simulink model "bus_roadtest_v3"  (R2018a)
settings: Solver=ode3  StartTime=0.0  StopTime=inf  FixedStep=0.01  RelTol=1e-3  EnableMultiTasking=on
PostLoadFcn:
  | , if any(exist('dsrtsu_mdlpostloadfcn', 'file') == [2, 3, 6]), try dsrtsu_mdlpostloadfcn('Execute', bdroot); catch fprintf('Error in PostLoadFcn (dsrtsu_mdlpostloadfcn) for model "%s":\n %s\n', bdroot, lasterr); end, end,
InitFcn:
  | bus_roadtest_v3_initial
values from neighbouring files (symbols this model uses):
  ay_max = 2    [Ini.m]
  delta_t = 0.01    [Ini.m]
  end_left_pass = 1    [Ini.m]
  end_right_pass = 0    [Ini.m]
  finish_node_id = length(Map_data(:,1))    [Ini.m]
  forward_length = 15    [Ini.m]
  gamma = sqrt(N_xaug+lambda)    [bus_roadtest_v3_initial.m]
  k_safe = 1    [Ini.m]
  nodes = nodes(1:index_node,:)    [Ini.m]
  rmin = 10    [Ini.m]
  segments = zeros(length(xy_ends_Pos(:,1)),3)    [Ini.m]
  start_node_id = 1    [Ini.m]
  Ts = 0.01    [bus_roadtest_v3_initial.m]
  Veh_CG = [0.5, 0.2]    [Ini.m]
  Veh_size = [1.99986,6.09558]    [Ini.m]
  vmax = 6    [Ini.m]
  weight = [weight_0,weight_0_cov,weight_i]    [bus_roadtest_v3_initial.m]
undefined symbols (not defined in the file or in its folder): Brake_table, DiscIntNeverNeededParam, Map_data, R, REF_GPS_RFS, Steer_gain_table, T
libraries: rtican x71, simulink x26, rti1401lib_adc_type4 x8, rti1401lib_dio_type4 x1
(part 7 of 18)

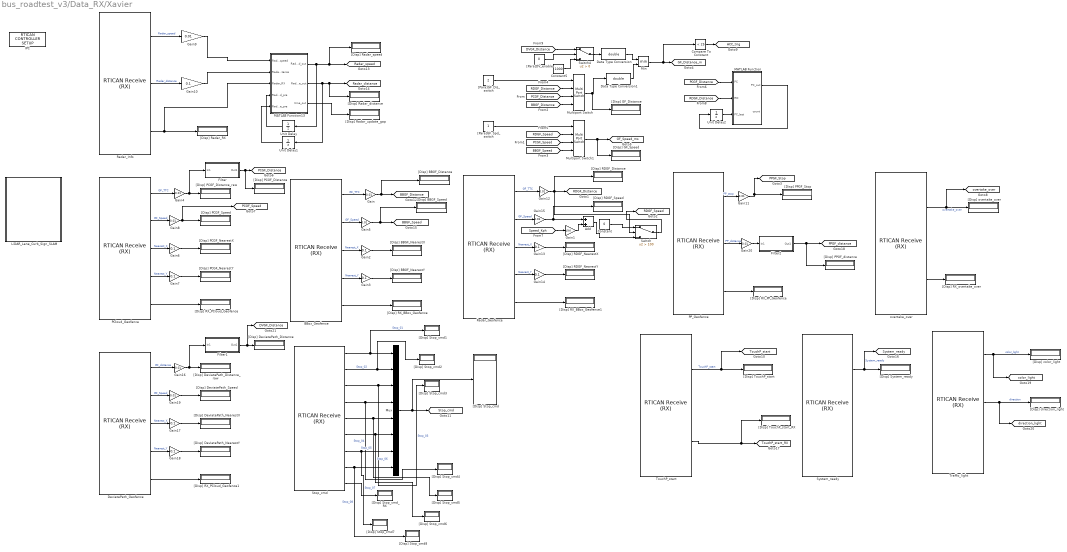
== system bus_roadtest_v3/Data_RX/Xavier ==
  Add : Sum
  BBox_Geofence : rtican/RTICAN Receive (RX)   Reserved1=[]  Reserved2=[]  Reserved3=[]  Reserved4=[]  SfcnMessage=[]  Msg_Struct=[]  BoardTypeNo=[]  BoardNo=[]  ChannelNo=[]  Parameters=[]  DialogFcn=[]  UnitName=[]  Revision=[]  UnitValues=[]  DSProperties=struct('RTI',struct('Version',uint32(5),'BlockType',struct('isSLSource',uint8(1),'isSLSink',uint8(1),'isHWSource',uint8(0),'isHWSink',uint8(0),'isSetup',uint8(0),'isInline',uint8(1),'isNonInline',uint8(0),'isInterrupt',uint8(0),'isChannelwise',uint8(0)),'IOBoardType','RTICAN','UnitType','MESSAGE','Identifier','RX','DialogType','MSVC','BlockSet','RTICAN','SlaveProcessor','CAN'))  RTIBlockInterface=struct('OutputPortsWidth',int32([1 1 1 1 1]),'OutputPortsActive',[1 1 1 1 1],'OutputPortsName',{{'GF_TTC','GF_Speed','Nearest_X','Nearest_Y',['RX status']}},'OutputPortsDataType',{{'SS_DOUBLE','SS_DOUBLE','SS_DOUBLE','SS_DOUBLE','SS_DOUBLE'}},'OutputPortsLabel',{{'GF_TTC','GF_Speed','Nearest_X','Nearest_Y',''}},'OutputPortsLabelMode','ON','InputPortsWidth',int32(0),'InputPortsActive',0,'DialogFcn','rtican_message_interface_gui','BlockDisplay',{{'','center'}},'IconTransparency','on','ParameterTunableNames',{{}},'InitLevel',3,'BlockName',struct('Token',{{'Geo_Fence_msg1'}}),'SampleTime',{{-1}},'TriggerPort',{{'none'}},'EnablePort',{{'none'}})  RTIBlockParameters=struct('BoardTypeNo',{{1,'OFF',[]}},'BoardNo',{{1,'ON',[1 16]}},'ChannelNo',{{1,'ON',[1 2]}},'Parameters',{{struct('DataFileSupport',struct('DataFileSelectedMaster',0,'DataFileSelectedLocal',0,'DataFileName',['<no datafile support>|'],'DataFileDate','','SelectedFile',['<no file selected>']),'Options',struct('StatusSelected',1,'TimeSelected',0,'DeltaTimeSelected',0,'BytePortSelected',0,'MessageLengthSelected',0,'TriggerPort',struct('Selected',0,'TriggerType',0),'UserCoding',struct('Selected',0,'InterfaceFile','UserDecodingFile','FcnName','UserDecodeFcn','InportSelected',0,'InportWidth',1,'OutportSelected',0,'OutportWidth',1),'EnablePortSelected',0,'SignalOnPortnameSelected',1,'UseRXService',0),'Message',struct('MsgOnBlocknameSelected',1,'MsgName','BBox_Geofence','MsgIdFormat',0,'MsgId',1425,'MsgLength',8,'NumSignals',4,'SampleTime',-1,'Signal',struct('SgnName',{'GF_TTC','GF_Speed','Nearest_X','Nearest_Y'},'SgnStartBit',{0,16,32,48},'SgnLength',{16,16,16,16},'SgnType',{0,0,0,0},'ModeValue',{-1,-1,-1,-1},'DataType',{1,1,1,1},'ByteLayout',{0,0,0,0},'Factor',{1,1,1,1},'Offset',{0,0,0,0},'SgnComment',{{''},{''},{''},{''}},'SgnUnit',{'','','',''},'Min',{0,0,0,0},'Max',{0,0,0,0},'SLDataType',{'SS_DOUBLE','SS_DOUBLE','SS_DOUBLE','SS_DOUBLE'}),'MsgIdNumFormat',1,'MsgComment',{{''}}),'Version',1.2,'general',struct('isFromLib',0)),'OFF',[]}},'GroupId',{{struct('Group',{{'RTICAN'}},'No',2,'Behavior',{{'NAMECHANGE'}},'BlockType',{{'SINK'}},'NameChangeFlag',0),'OFF',[]}},'SFcnRTICANMessage',{{struct('MsgType','RX','SFcnPortType','Scalar','MsgName','BBox_Geofence','MsgIdFormat','STD','MsgId',1425,'MsgLength',8,'NumSignals',4,'SampleTime',-1,'Signal',struct('SgnName',{'GF_TTC','GF_Speed','Nearest_X','Nearest_Y'},'SgnStartBit',{0,16,32,48},'SgnLength',{16,16,16,16},'SgnType',{'standard','standard','standard','standard'},'ModeValue',{-1,-1,-1,-1},'DataType',{['signed int'],['signed int'],['signed int'],['signed int']},'ByteLayout',{['little endian'],['little endian'],['little endian'],['little endian']},'Factor',{1,1,1,1},'Offset',{0,0,0,0},'SLDataType',{'SS_DOUBLE','SS_DOUBLE','SS_DOUBLE','SS_DOUBLE'}),'StatusSelected','yes','TimeSelected','no','DeltaTimeSelected','no','BytePortSelected','no','MessageLengthSelected','no','TriggerPort',struct('Selected','no','TriggerType',0),'UserCoding',struct('Selected','no','InterfaceFile','UserDecodingFile','FcnName','UserDecodeFcn','InportSelected','no','InportWidth',1,'OutportSelected','no','OutportWidth',1),'EnablePortSelected','no','UseRXService','no','BoardType','DS1','BoardNo',1,'ControllerNo',1),'OFF',[]}},'TLCFileName',{{'rtican_rx_message','OFF',[]}})  RTISFcnParameters=struct('SFcnRTICANMessage','struct','TLCFileName','char')  RTIBlockParaDefault=struct('BoardTypeNo',4302,'BoardNo',1,'ChannelNo',1,'Parameters',struct('DataFileSupport',struct('DataFileSelectedMaster',0,'DataFileSelectedLocal',0,'DataFileName','','DataFileDate','','SelectedFile',['<no file selected>']),'Options',struct('StatusSelected',1,'TimeSelected',1,'DeltaTimeSelected',1,'BytePortSelected',0,'MessageLengthSelected',0,'TriggerPort',struct('Selected',0,'TriggerType','rising'),'UserCoding',struct('Selected',0,'InterfaceFile','UserDecodingFile','FcnName','UserDecodeFcn','InportSelected',0,'InportWidth',1,'OutportSelected',0,'OutportWidth',1),'EnablePortSelected',0,'SignalOnPortnameSelected',1,'UseRXService',0),'Message',struct('MsgOnBlocknameSelected',0,'MsgName',['RX Message'],'MsgIdFormat',0,'MsgId',100,'MsgLength',8,'NumSignals',1,'SampleTime',-1,'Signal',struct('SgnName',['RX signal'],'SgnStartBit',0,'SgnLength',8,'SgnType',0,'ModeValue',-1,'DataType',0,'SLDataType','SS_DOUBLE','ByteLayout',0,'Factor',1,'Offset',0,'Min',0,'Max',255,'SgnComment',{{}},'SgnUnit',''),'MsgIdNumFormat',0,'MsgComment',{{''}}),'Version',1.2,'general',struct('isFromLib',1)),'GroupId',struct('Group',{{'RTICAN'}},'No',1,'Behavior',{{'NAMECHANGE'}},'BlockType',{{'SINK'}},'NameChangeFlag',0),'SFcnRTICANMessage',struct('MsgType','RX','MsgName',['RX Message'],'MsgIdFormat','STD','MsgId',100,'MsgLength',8,'NumSignals',1,'SampleTime',-1,'Signal',struct('SgnName',['RX signal'],'SgnStartBit',0,'SgnLength',8,'SgnType','standard','ModeValue',-1,'DataType',['unsigned int'],'ByteLayout',['little endian'],'SLDataType','SS_DOUBLE','Factor',1,'Offset',0),'StatusSelected','yes','TimeSelected','yes','DeltaTimeSelected','yes','BytePortSelected','no','MessageLengthSelected','no','EnablePortSelected','no','UserCoding',struct('Selected','no','InterfaceFile','UserDecodingFile','FcnName','UserDecodeFcn','InportSelected','no','InportWidth',1,'OutportSelected','no','OutportWidth',1),'TriggerPort',struct('Selected','no','TriggerType','rising'),'UseRXService','no','BoardType','DS4302','BoardNo',1,'ControllerNo',1,'SFcnPortType','Scalar'),'TLCFileName','rtican_rx_message')
      settings: AttributesFormatString=Group Id: RTICAN2\n  SourceProductName=dSPACE RTI CAN Blockset
  Compare To Constant : simulink/Logic and Bit Operations/Compare To Constant  relop=<  const=25  OutDataTypeStr=uint8
  Constant : Constant  Value=0
  Constant5 : Constant  Value=1000
  Data Type Conversion : DataTypeConversion  OutDataTypeStr=double
  Data Type Conversion1 : DataTypeConversion  OutDataTypeStr=double
  DeviatePath_Geofence : rtican/RTICAN Receive (RX)   Reserved1=[]  Reserved2=[]  Reserved3=[]  Reserved4=[]  SfcnMessage=[]  Msg_Struct=[]  BoardTypeNo=[]  BoardNo=[]  ChannelNo=[]  Parameters=[]  DialogFcn=[]  UnitName=[]  Revision=[]  UnitValues=[]  DSProperties=struct('RTI',struct('Version',uint32(5),'BlockType',struct('isSLSource',uint8(1),'isSLSink',uint8(1),'isHWSource',uint8(0),'isHWSink',uint8(0),'isSetup',uint8(0),'isInline',uint8(1),'isNonInline',uint8(0),'isInterrupt',uint8(0),'isChannelwise',uint8(0)),'IOBoardType','RTICAN','UnitType','MESSAGE','Identifier','RX','DialogType','MSVC','BlockSet','RTICAN','SlaveProcessor','CAN'))  RTIBlockInterface=struct('OutputPortsWidth',int32([1 1 1 1 1]),'OutputPortsActive',[1 1 1 1 1],'OutputPortsName',{{'GF_distance','GF_Speed','Nearest_X','Nearest_Y',['RX status']}},'OutputPortsDataType',{{'SS_DOUBLE','SS_DOUBLE','SS_DOUBLE','SS_DOUBLE','SS_DOUBLE'}},'OutputPortsLabel',{{'GF_distance','GF_Speed','Nearest_X','Nearest_Y',''}},'OutputPortsLabelMode','ON','InputPortsWidth',int32(0),'InputPortsActive',0,'DialogFcn','rtican_message_interface_gui','BlockDisplay',{{'','center'}},'IconTransparency','on','ParameterTunableNames',{{}},'InitLevel',3,'BlockName',struct('Token',{{'DeviatePath_Geofence'}}),'SampleTime',{{-1}},'TriggerPort',{{'none'}},'EnablePort',{{'none'}})  RTIBlockParameters=struct('BoardTypeNo',{{1,'OFF',[]}},'BoardNo',{{1,'ON',[1 16]}},'ChannelNo',{{1,'ON',[1 2]}},'Parameters',{{struct('DataFileSupport',struct('DataFileSelectedMaster',0,'DataFileSelectedLocal',0,'DataFileName',['<no datafile support>|'],'DataFileDate','','SelectedFile',['<no file selected>']),'Options',struct('StatusSelected',1,'TimeSelected',0,'DeltaTimeSelected',0,'BytePortSelected',0,'MessageLengthSelected',0,'TriggerPort',struct('Selected',0,'TriggerType',0),'UserCoding',struct('Selected',0,'InterfaceFile','UserDecodingFile','FcnName','UserDecodeFcn','InportSelected',0,'InportWidth',1,'OutportSelected',0,'OutportWidth',1),'EnablePortSelected',0,'SignalOnPortnameSelected',1,'UseRXService',0),'Message',struct('MsgOnBlocknameSelected',1,'MsgName','DeviatePath_Geofence','MsgIdFormat',0,'MsgId',1427,'MsgLength',8,'NumSignals',4,'SampleTime',-1,'Signal',struct('SgnName',{'GF_distance','GF_Speed','Nearest_X','Nearest_Y'},'SgnStartBit',{0,16,32,48},'SgnLength',{16,16,16,16},'SgnType',{0,0,0,0},'ModeValue',{-1,-1,-1,-1},'DataType',{1,1,1,1},'ByteLayout',{0,0,0,0},'Factor',{1,1,1,1},'Offset',{0,0,0,0},'SgnComment',{{''},{''},{''},{''}},'SgnUnit',{'','','',''},'Min',{0,0,0,0},'Max',{0,0,0,0},'SLDataType',{'SS_DOUBLE','SS_DOUBLE','SS_DOUBLE','SS_DOUBLE'}),'MsgIdNumFormat',1,'MsgComment',{{''}}),'Version',1.2,'general',struct('isFromLib',0)),'OFF',[]}},'GroupId',{{struct('Group',{{'RTICAN'}},'No',2,'Behavior',{{'NAMECHANGE'}},'BlockType',{{'SINK'}},'NameChangeFlag',0),'OFF',[]}},'SFcnRTICANMessage',{{struct('MsgType','RX','SFcnPortType','Scalar','MsgName','DeviatePath_Geofence','MsgIdFormat','STD','MsgId',1427,'MsgLength',8,'NumSignals',4,'SampleTime',-1,'Signal',struct('SgnName',{'GF_distance','GF_Speed','Nearest_X','Nearest_Y'},'SgnStartBit',{0,16,32,48},'SgnLength',{16,16,16,16},'SgnType',{'standard','standard','standard','standard'},'ModeValue',{-1,-1,-1,-1},'DataType',{['signed int'],['signed int'],['signed int'],['signed int']},'ByteLayout',{['little endian'],['little endian'],['little endian'],['little endian']},'Factor',{1,1,1,1},'Offset',{0,0,0,0},'SLDataType',{'SS_DOUBLE','SS_DOUBLE','SS_DOUBLE','SS_DOUBLE'}),'StatusSelected','yes','TimeSelected','no','DeltaTimeSelected','no','BytePortSelected','no','MessageLengthSelected','no','TriggerPort',struct('Selected','no','TriggerType',0),'UserCoding',struct('Selected','no','InterfaceFile','UserDecodingFile','FcnName','UserDecodeFcn','InportSelected','no','InportWidth',1,'OutportSelected','no','OutportWidth',1),'EnablePortSelected','no','UseRXService','no','BoardType','DS1','BoardNo',1,'ControllerNo',1),'OFF',[]}},'TLCFileName',{{'rtican_rx_message','OFF',[]}})  RTISFcnParameters=struct('SFcnRTICANMessage','struct','TLCFileName','char')  RTIBlockParaDefault=struct('BoardTypeNo',4302,'BoardNo',1,'ChannelNo',1,'Parameters',struct('DataFileSupport',struct('DataFileSelectedMaster',0,'DataFileSelectedLocal',0,'DataFileName','','DataFileDate','','SelectedFile',['<no file selected>']),'Options',struct('StatusSelected',1,'TimeSelected',1,'DeltaTimeSelected',1,'BytePortSelected',0,'MessageLengthSelected',0,'TriggerPort',struct('Selected',0,'TriggerType','rising'),'UserCoding',struct('Selected',0,'InterfaceFile','UserDecodingFile','FcnName','UserDecodeFcn','InportSelected',0,'InportWidth',1,'OutportSelected',0,'OutportWidth',1),'EnablePortSelected',0,'SignalOnPortnameSelected',1,'UseRXService',0),'Message',struct('MsgOnBlocknameSelected',0,'MsgName',['RX Message'],'MsgIdFormat',0,'MsgId',100,'MsgLength',8,'NumSignals',1,'SampleTime',-1,'Signal',struct('SgnName',['RX signal'],'SgnStartBit',0,'SgnLength',8,'SgnType',0,'ModeValue',-1,'DataType',0,'SLDataType','SS_DOUBLE','ByteLayout',0,'Factor',1,'Offset',0,'Min',0,'Max',255,'SgnComment',{{}},'SgnUnit',''),'MsgIdNumFormat',0,'MsgComment',{{''}}),'Version',1.2,'general',struct('isFromLib',1)),'GroupId',struct('Group',{{'RTICAN'}},'No',1,'Behavior',{{'NAMECHANGE'}},'BlockType',{{'SINK'}},'NameChangeFlag',0),'SFcnRTICANMessage',struct('MsgType','RX','MsgName',['RX Message'],'MsgIdFormat','STD','MsgId',100,'MsgLength',8,'NumSignals',1,'SampleTime',-1,'Signal',struct('SgnName',['RX signal'],'SgnStartBit',0,'SgnLength',8,'SgnType','standard','ModeValue',-1,'DataType',['unsigned int'],'ByteLayout',['little endian'],'SLDataType','SS_DOUBLE','Factor',1,'Offset',0),'StatusSelected','yes','TimeSelected','yes','DeltaTimeSelected','yes','BytePortSelected','no','MessageLengthSelected','no','EnablePortSelected','no','UserCoding',struct('Selected','no','InterfaceFile','UserDecodingFile','FcnName','UserDecodeFcn','InportSelected','no','InportWidth',1,'OutportSelected','no','OutportWidth',1),'TriggerPort',struct('Selected','no','TriggerType','rising'),'UseRXService','no','BoardType','DS4302','BoardNo',1,'ControllerNo',1,'SFcnPortType','Scalar'),'TLCFileName','rtican_rx_message')
      settings: AttributesFormatString=Group Id: RTICAN2\n  SourceProductName=dSPACE RTI CAN Blockset
  Filter : Subsystem
  Filter1 : Subsystem
  Filter2 : Subsystem
  Gain{,4..5,8..9,11..12,15..16,19..20} (11 alike) : Gain  Gain=0.01
  Gain1 : Gain  Gain=1/3.6
  Gain{2..3,6..7,10,13..14,17..18} (9 alike) : Gain  Gain=0.1
  IPC : rtican/RTICAN CONTROLLER SETUP   Reserved1=[]  Reserved2=[]  Reserved3=[]  Reserved4=[]  AcceptanceMask=[]  ArbitrationField=[]  Parameters=[]  SFcnRTICANSettings=[]  MS_Struct=[]  BoardTypeNo=[]  BoardNo=[]  ChannelNo=[]  DialogFcn=[]  UnitName=[]  Revision=[]  UnitValues=[]  DSProperties=struct('RTI',struct('Version',uint32(12),'BlockType',struct('isSLSource',uint8(0),'isSLSink',uint8(0),'isHWSource',uint8(0),'isHWSink',uint8(0),'isSetup',uint8(1),'isInline',uint8(1),'isNonInline',uint8(0),'isInterrupt',uint8(0),'isChannelwise',uint8(0)),'IOBoardType','RTICAN','UnitType','NON_MESSAGE','Identifier','MASTER','DialogType','ML','BlockSet','RTICAN','SlaveProcessor','CAN'))  RTIBlockInterface=struct('InputPortsWidth',int32(0),'InputPortsActive',0,'OutputPortsWidth',int32(0),'OutputPortsActive',0,'DialogFcn','rtican_master_setup_gui','BlockDisplay',{{['CAN CONTROLLER\n SETUP'],'center'}},'IconTransparency','on','InitLevel',3,'IWork',{{{'',uint32(2)}}},'BlockName',struct('Token',{{'CAN_TYPE','_SETUP_M','_C'}},'BlockParam',{{'BoardTypeNo','BoardNo','ChannelNo'}}),'ParameterTunableNames',{{}})  RTIBlockParameters="struct('BoardTypeNo',{{1,'OFF',[]}},'BoardNo',{{1,'ON',[1 16]}},'ChannelNo',{{1,'ON',[1 2]}},'AcceptanceMask',{{0,'OFF',[]}},'ArbitrationField',{{0,'OFF',[]}},'Parameters',{{struct('Config',struct('Baudrate',500,'SampleMode',1,'UsedParamSet',1,'validSettings',1,'isBTRvalues',0,'Advanced',struct('Baudrate',{500,500,500},'Frequency',{24000000,36000000,64000000},'Settings',{struct('SMPL',0,'BRP',0,'NBT',24,'TSEG1',15,'TSEG2',6,'SJW',3,'SP',70),struct('SMPL',0,'BRP',1,'NBT',18,'TSEG1',14,'TSEG2',1,'SJW',1,'SP',88),struct('SMPL',0,'BRP',3,'NBT',16,'TSEG1',12,'TSEG2',1,'SJW',1,'SP',87)},'BTR0',{192,65,67},'BTR1',{111,30,28})),'configType',1,'Options',struct('DataFileSelected',0,'DataFileName',{{['<no datafile support>']}},'DataFileDate',{{''}},'InterfaceFcn','rtican_dbc_file_parser','InterfaceFcnFileName','','LabelConfigType','volatile','AcceptanceMaskSelected',0,'MsgDataType','AllwaysDouble','NumType','hex','MaskType','STD','AcceptanceMask',0,'ArbitrationField',0,'UseMultipleMessageAccess',0),'RxReceiveStdOptions',struct('RxServiceStdEnabled',0,'RxServiceStdMsgIdent',1000,'RxServiceStdIdentNumType',1,'RxServiceStdIdentMask',0,'RxServiceStdMaskNumType',1,'RxServiceStdQueueSize',64),'RxReceiveXtdOptions',struct('RxServiceXtdEnabled',0,'RxServiceXtdMsgIdent',1001,'RxServiceXtdIdentNumType',1,'RxServiceXtdIdentMask',0,'RxServiceXtdMaskNumType',1,'RxServiceXtdQueueSize',64),'PartialNetworkingOptions',struct('switchedon',0,'format',1,'idmask',['    XXXXX XXXXXXXX XXXXXXXX XXXXXXXX'],'idcode','0','idfilter','0','datamaskused',0,'datalength',1,'datamask','0x0000000000000000','partialnetworkenable',0),'general',struct('Termination_common',1,'Termination_C252',1,'BusConfigurationRegister',0,'Transceiver','ISO11898','isFromLib',0)),'OFF',[]}},'CCPParameters',{{struct('CRO',struct('Format','STD','NumFormat','hex','Id',1639),'DTO',struct('Format','STD','NumFormat','hex','Id',2017),'StationAdr',struct('NumFormat','hex','Value',57),'StationId',struct('Value',['dSPACE CCP Service']),'Enabled',0),'OFF',[]}},'XCPParameters',{{struct('MASTER',struct('Format','STD','NumFormat','hex','Id',256),'SLAVE',struct('Format','STD','NumFormat','hex','Id',510),'Enabled',0,'PIDTransmissionEnabled',0),'OFF',[]}},'GroupId',{{struct('Group',{{'RTICAN'}},'No',2,'Behavior',{{'EVER'}},'BlockType',{{'SOURCE'}},'NameChangeFlag',1),'OFF',[]}},'SFcnRTICANSettings',{{struct('Baudrate',500,'configType',1,'AdvancedConfig',struct('Frequency',{},'BTR0',{},'BTR1',{}),'UsedParamSet',1,'STDMaskSelected','no','XTDMaskSelected','no','BoardType','DS1','BoardNo',1,'ControllerNo',1,'Transceiver','ISO11898','BusConfigRegister',0,'TerminationRes',120,'UseMultipleMessageAccess','no','STDRXSrvcUsed','no','STDRXSrvcMsgId',1000,'STDRXSrvcMsgMask',0,'STDRXSrvcQueueSize',64,'XTDRXSrvcUsed','no','XTDRXSrvcMsgId',1001,'XTDRXSrvcQueueSize',64,'XTDRXSrvcMsgMask',0,'PN_IsPNTransciever',0,'PN_IsPNEnabled',0,'PN_MsgFormat',1,'PN_idcode',0,'PN_idmask',2047,'PN_datamaskused',0,'PN_datalength',0,'PN_datamask',['0xFF, 0xFF, 0xFF, 0xFF, 0xFF, 0xFF, 0xFF, 0xFF']),'OFF',[]}},'SFcnRTICCPSettings',{{struct('CRO',struct('Format','STD','NumFormat','hex','Id',1639),'DTO',struct('Format','STD','NumFormat','hex','Id',2017),'StationAdr',struct('NumFormat','hex','Value',57),'StationId',struct('Value',['dSPACE CCP Service']),'Enabled',0),'OFF',[]}},'SFcnRTIXCPSettings',{{struct('MASTER',struct('Format','STD','NumFormat','hex','Id',256),'SLAVE',struct('Format','STD','NumFormat','hex','Id',510),'Enabled',0,'PIDTransmissionEnabled',0),'OFF',[]}},'TLCFileName',{{'rtican_master_setup','OFF',[]}})"  RTISFcnParameters=struct('SFcnRTICANSettings','struct','SFcnRTICCPSettings','struct','SFcnRTIXCPSettings','struct','AcceptanceMask','int32','ArbitrationField','int32','TLCFileName','char')  RTIBlockParaDefault="struct('BoardTypeNo',4302,'BoardNo',1,'ChannelNo',1,'AcceptanceMask',0,'ArbitrationField',0,'Parameters',struct('Config',struct('Baudrate',500,'SampleMode',1,'UsedParamSet',1,'validSettings',1,'isBTRvalues',0,'Advanced',struct('Frequency',16000000,'BTR0',64,'BTR1',28,'Settings',struct('SMPL',0,'BRP',0,'NBT',16,'TSEG1',12,'TSEG2',1,'SJW',1,'SP',87))),'configType',1,'Options',struct('DataFileSelected',0,'DataFileName',{{['<no datafile support>']}},'DataFileDate',{{''}},'InterfaceFcn','rtican_dbc_file_parser','InterfaceFcnFileName','','LabelConfigType','volatile','AcceptanceMaskSelected',0,'MsgDataType','AllwaysDouble','NumType','hex','MaskType','STD','AcceptanceMask',0,'ArbitrationField',0,'UseMultipleMessageAccess',0),'RxReceiveStdOptions',struct('RxServiceStdEnabled',0,'RxServiceStdMsgIdent',1000,'RxServiceStdIdentNumType',1,'RxServiceStdIdentMask',0,'RxServiceStdMaskNumType',1,'RxServiceStdQueueSize',64),'RxReceiveXtdOptions',struct('RxServiceXtdEnabled',0,'RxServiceXtdMsgIdent',1001,'RxServiceXtdIdentNumType',1,'RxServiceXtdIdentMask',0,'RxServiceXtdMaskNumType',1,'RxServiceXtdQueueSize',64),'PartialNetworkingOptions',struct('switchedon',0,'format',1,'idmask',['    XXXXX XXXXXXXX XXXXXXXX XXXXXXXX'],'idcode','0','idfilter','0','datamaskused',0,'datalength',1,'datamask','0x0000000000000000','partialnetworkenable',0),'general',struct('Termination_common',1,'Termination_C252',1,'BusConfigurationRegister',0,'Transceiver','ISO11898','isFromLib',1)),'CCPParameters',struct('CRO',struct('Format','STD','NumFormat','hex','Id',1639),'DTO',struct('Format','STD','NumFormat','hex','Id',2017),'StationAdr',struct('NumFormat','hex','Value',57),'StationId',struct('Value',['dSPACE CCP Service']),'Enabled',0),'XCPParameters',struct('MASTER',struct('Format','STD','NumFormat','hex','Id',256),'SLAVE',struct('Format','STD','NumFormat','hex','Id',510),'Enabled',0,'PIDTransmissionEnabled',0),'GroupId',struct('Group',{{'RTICAN'}},'No',1,'Behavior',{{'EVER'}},'BlockType',{{'SOURCE'}},'NameChangeFlag',1),'SFcnRTICANSettings',struct('Baudrate',500,'configType',1,'AdvandedConfig',struct('Frequency',16000000,'BTR0','0x40','BTR1','0x1C'),'UsedParamSet',1,'STDMaskSelected','no','XTDMaskSelected','no','BoardType','DS4302','BoardNo',1,'ControllerNo',1,'Transceiver','ISO11898','BusConfigRegister',0,'TerminationRes',120,'UseMultipleMessageAccess','no','STDRXSrvcUsed','no','STDRXSrvcMsgId',1000,'STDRXSrvcMsgMask',0,'STDRXSrvcQueueSize',64,'XTDRXSrvcUsed','no','XTDRXSrvcMsgId',1001,'XTDRXSrvcQueueSize',64,'XTDRXSrvcMsgMask',0),'SFcnRTICCPSettings',struct('CRO',struct('Format','STD','NumFormat','hex','Id',1639),'DTO',struct('Format','STD','NumFormat','hex','Id',2017),'StationAdr',struct('NumFormat','hex','Value',57),'StationId',struct('Value',['dSPACE CCP Service']),'Enabled',0),'SFcnRTIXCPSettings',struct('MASTER',struct('Format','STD','NumFormat','hex','Id',256),'SLAVE',struct('Format','STD','NumFormat','hex','Id',510),'Enabled',0,'PIDTransmissionEnabled',0),'TLCFileName','rtican_master_setup')"
      settings: AttributesFormatString=Group Id: RTICAN2\n  SourceProductName=dSPACE RTI CAN Blockset
  LiDAR_Lane_Curb_Sign_SLAM : Subsystem
  MATLAB Function : MATLAB Function  TreatAsAtomicUnit=on
  MATLAB Function13 : MATLAB Function  TreatAsAtomicUnit=on
  Min : MinMax  Inputs=2
  Multiport Switch : MultiPortSwitch  DataPortOrder=Specify indices
  Multiport Switch1 : MultiPortSwitch  DataPortOrder=Specify indices
  Mux : Mux  Inputs=8
  PCloud_Geofence : rtican/RTICAN Receive (RX)   Reserved1=[]  Reserved2=[]  Reserved3=[]  Reserved4=[]  SfcnMessage=[]  Msg_Struct=[]  BoardTypeNo=[]  BoardNo=[]  ChannelNo=[]  Parameters=[]  DialogFcn=[]  UnitName=[]  Revision=[]  UnitValues=[]  DSProperties=struct('RTI',struct('Version',uint32(5),'BlockType',struct('isSLSource',uint8(1),'isSLSink',uint8(1),'isHWSource',uint8(0),'isHWSink',uint8(0),'isSetup',uint8(0),'isInline',uint8(1),'isNonInline',uint8(0),'isInterrupt',uint8(0),'isChannelwise',uint8(0)),'IOBoardType','RTICAN','UnitType','MESSAGE','Identifier','RX','DialogType','MSVC','BlockSet','RTICAN','SlaveProcessor','CAN'))  RTIBlockInterface=struct('OutputPortsWidth',int32([1 1 1 1 1]),'OutputPortsActive',[1 1 1 1 1],'OutputPortsName',{{'GF_TTC','GF_Speed','Nearest_X','Nearest_Y',['RX status']}},'OutputPortsDataType',{{'SS_DOUBLE','SS_DOUBLE','SS_DOUBLE','SS_DOUBLE','SS_DOUBLE'}},'OutputPortsLabel',{{'GF_TTC','GF_Speed','Nearest_X','Nearest_Y',''}},'OutputPortsLabelMode','ON','InputPortsWidth',int32(0),'InputPortsActive',0,'DialogFcn','rtican_message_interface_gui','BlockDisplay',{{'','center'}},'IconTransparency','on','ParameterTunableNames',{{}},'InitLevel',3,'BlockName',struct('Token',{{'PCloud_Geofence'}}),'SampleTime',{{-1}},'TriggerPort',{{'none'}},'EnablePort',{{'none'}})  RTIBlockParameters=struct('BoardTypeNo',{{1,'OFF',[]}},'BoardNo',{{1,'ON',[1 16]}},'ChannelNo',{{1,'ON',[1 2]}},'Parameters',{{struct('DataFileSupport',struct('DataFileSelectedMaster',0,'DataFileSelectedLocal',0,'DataFileName',['<no datafile support>|'],'DataFileDate','','SelectedFile',['<no file selected>']),'Options',struct('StatusSelected',1,'TimeSelected',0,'DeltaTimeSelected',0,'BytePortSelected',0,'MessageLengthSelected',0,'TriggerPort',struct('Selected',0,'TriggerType',0),'UserCoding',struct('Selected',0,'InterfaceFile','UserDecodingFile','FcnName','UserDecodeFcn','InportSelected',0,'InportWidth',1,'OutportSelected',0,'OutportWidth',1),'EnablePortSelected',0,'SignalOnPortnameSelected',1,'UseRXService',0),'Message',struct('MsgOnBlocknameSelected',1,'MsgName','PCloud_Geofence','MsgIdFormat',0,'MsgId',1424,'MsgLength',8,'NumSignals',4,'SampleTime',-1,'Signal',struct('SgnName',{'GF_TTC','GF_Speed','Nearest_X','Nearest_Y'},'SgnStartBit',{0,16,32,48},'SgnLength',{16,16,16,16},'SgnType',{0,0,0,0},'ModeValue',{-1,-1,-1,-1},'DataType',{1,1,1,1},'ByteLayout',{0,0,0,0},'Factor',{1,1,1,1},'Offset',{0,0,0,0},'SgnComment',{{''},{''},{''},{''}},'SgnUnit',{'','','',''},'Min',{0,0,0,0},'Max',{0,0,0,0},'SLDataType',{'SS_DOUBLE','SS_DOUBLE','SS_DOUBLE','SS_DOUBLE'}),'MsgIdNumFormat',1,'MsgComment',{{''}}),'Version',1.2,'general',struct('isFromLib',0)),'OFF',[]}},'GroupId',{{struct('Group',{{'RTICAN'}},'No',2,'Behavior',{{'NAMECHANGE'}},'BlockType',{{'SINK'}},'NameChangeFlag',0),'OFF',[]}},'SFcnRTICANMessage',{{struct('MsgType','RX','SFcnPortType','Scalar','MsgName','PCloud_Geofence','MsgIdFormat','STD','MsgId',1424,'MsgLength',8,'NumSignals',4,'SampleTime',-1,'Signal',struct('SgnName',{'GF_TTC','GF_Speed','Nearest_X','Nearest_Y'},'SgnStartBit',{0,16,32,48},'SgnLength',{16,16,16,16},'SgnType',{'standard','standard','standard','standard'},'ModeValue',{-1,-1,-1,-1},'DataType',{['signed int'],['signed int'],['signed int'],['signed int']},'ByteLayout',{['little endian'],['little endian'],['little endian'],['little endian']},'Factor',{1,1,1,1},'Offset',{0,0,0,0},'SLDataType',{'SS_DOUBLE','SS_DOUBLE','SS_DOUBLE','SS_DOUBLE'}),'StatusSelected','yes','TimeSelected','no','DeltaTimeSelected','no','BytePortSelected','no','MessageLengthSelected','no','TriggerPort',struct('Selected','no','TriggerType',0),'UserCoding',struct('Selected','no','InterfaceFile','UserDecodingFile','FcnName','UserDecodeFcn','InportSelected','no','InportWidth',1,'OutportSelected','no','OutportWidth',1),'EnablePortSelected','no','UseRXService','no','BoardType','DS1','BoardNo',1,'ControllerNo',1),'OFF',[]}},'TLCFileName',{{'rtican_rx_message','OFF',[]}})  RTISFcnParameters=struct('SFcnRTICANMessage','struct','TLCFileName','char')  RTIBlockParaDefault=struct('BoardTypeNo',4302,'BoardNo',1,'ChannelNo',1,'Parameters',struct('DataFileSupport',struct('DataFileSelectedMaster',0,'DataFileSelectedLocal',0,'DataFileName','','DataFileDate','','SelectedFile',['<no file selected>']),'Options',struct('StatusSelected',1,'TimeSelected',1,'DeltaTimeSelected',1,'BytePortSelected',0,'MessageLengthSelected',0,'TriggerPort',struct('Selected',0,'TriggerType','rising'),'UserCoding',struct('Selected',0,'InterfaceFile','UserDecodingFile','FcnName','UserDecodeFcn','InportSelected',0,'InportWidth',1,'OutportSelected',0,'OutportWidth',1),'EnablePortSelected',0,'SignalOnPortnameSelected',1,'UseRXService',0),'Message',struct('MsgOnBlocknameSelected',0,'MsgName',['RX Message'],'MsgIdFormat',0,'MsgId',100,'MsgLength',8,'NumSignals',1,'SampleTime',-1,'Signal',struct('SgnName',['RX signal'],'SgnStartBit',0,'SgnLength',8,'SgnType',0,'ModeValue',-1,'DataType',0,'SLDataType','SS_DOUBLE','ByteLayout',0,'Factor',1,'Offset',0,'Min',0,'Max',255,'SgnComment',{{}},'SgnUnit',''),'MsgIdNumFormat',0,'MsgComment',{{''}}),'Version',1.2,'general',struct('isFromLib',1)),'GroupId',struct('Group',{{'RTICAN'}},'No',1,'Behavior',{{'NAMECHANGE'}},'BlockType',{{'SINK'}},'NameChangeFlag',0),'SFcnRTICANMessage',struct('MsgType','RX','MsgName',['RX Message'],'MsgIdFormat','STD','MsgId',100,'MsgLength',8,'NumSignals',1,'SampleTime',-1,'Signal',struct('SgnName',['RX signal'],'SgnStartBit',0,'SgnLength',8,'SgnType','standard','ModeValue',-1,'DataType',['unsigned int'],'ByteLayout',['little endian'],'SLDataType','SS_DOUBLE','Factor',1,'Offset',0),'StatusSelected','yes','TimeSelected','yes','DeltaTimeSelected','yes','BytePortSelected','no','MessageLengthSelected','no','EnablePortSelected','no','UserCoding',struct('Selected','no','InterfaceFile','UserDecodingFile','FcnName','UserDecodeFcn','InportSelected','no','InportWidth',1,'OutportSelected','no','OutportWidth',1),'TriggerPort',struct('Selected','no','TriggerType','rising'),'UseRXService','no','BoardType','DS4302','BoardNo',1,'ControllerNo',1,'SFcnPortType','Scalar'),'TLCFileName','rtican_rx_message')
      settings: AttributesFormatString=Group Id: RTICAN2\n  SourceProductName=dSPACE RTI CAN Blockset
  PP_Geofence : rtican/RTICAN Receive (RX)   Reserved1=[]  Reserved2=[]  Reserved3=[]  Reserved4=[]  SfcnMessage=[]  Msg_Struct=[]  BoardTypeNo=[]  BoardNo=[]  ChannelNo=[]  Parameters=[]  DialogFcn=[]  UnitName=[]  Revision=[]  UnitValues=[]  DSProperties=struct('RTI',struct('Version',uint32(5),'BlockType',struct('isSLSource',uint8(1),'isSLSink',uint8(1),'isHWSource',uint8(0),'isHWSink',uint8(0),'isSetup',uint8(0),'isInline',uint8(1),'isNonInline',uint8(0),'isInterrupt',uint8(0),'isChannelwise',uint8(0)),'IOBoardType','RTICAN','UnitType','MESSAGE','Identifier','RX','DialogType','MSVC','BlockSet','RTICAN','SlaveProcessor','CAN'))  RTIBlockInterface=struct('OutputPortsWidth',int32([1 1 1]),'OutputPortsActive',[1 1 1],'OutputPortsName',{{'PP_stop','PP_distance',['RX status']}},'OutputPortsDataType',{{'SS_DOUBLE','SS_DOUBLE','SS_DOUBLE'}},'OutputPortsLabel',{{'PP_stop','PP_distance',''}},'OutputPortsLabelMode','ON','InputPortsWidth',int32(0),'InputPortsActive',0,'DialogFcn','rtican_message_interface_gui','BlockDisplay',{{'','center'}},'IconTransparency','on','ParameterTunableNames',{{}},'InitLevel',3,'BlockName',struct('Token',{{'Geo_Fence_msg1'}}),'SampleTime',{{-1}},'TriggerPort',{{'none'}},'EnablePort',{{'none'}})  RTIBlockParameters=struct('BoardTypeNo',{{1,'OFF',[]}},'BoardNo',{{1,'ON',[1 16]}},'ChannelNo',{{1,'ON',[1 2]}},'Parameters',{{struct('DataFileSupport',struct('DataFileSelectedMaster',0,'DataFileSelectedLocal',0,'DataFileName',['<no datafile support>|'],'DataFileDate','','SelectedFile',['<no file selected>']),'Options',struct('StatusSelected',1,'TimeSelected',0,'DeltaTimeSelected',0,'BytePortSelected',0,'MessageLengthSelected',0,'TriggerPort',struct('Selected',0,'TriggerType',0),'UserCoding',struct('Selected',0,'InterfaceFile','UserDecodingFile','FcnName','UserDecodeFcn','InportSelected',0,'InportWidth',1,'OutportSelected',0,'OutportWidth',1),'EnablePortSelected',0,'SignalOnPortnameSelected',1,'UseRXService',0),'Message',struct('MsgOnBlocknameSelected',1,'MsgName','PP_Geofence','MsgIdFormat',0,'MsgId',1429,'MsgLength',8,'NumSignals',2,'SampleTime',-1,'Signal',struct('SgnName',{'PP_stop','PP_distance'},'SgnStartBit',{0,16},'SgnLength',{16,16},'SgnType',{0,0},'ModeValue',{-1,-1},'DataType',{1,1},'ByteLayout',{0,0},'Factor',{1,1},'Offset',{0,0},'SgnComment',{{''},{''}},'SgnUnit',{'',''},'Min',{0,0},'Max',{0,0},'SLDataType',{'SS_DOUBLE','SS_DOUBLE'}),'MsgIdNumFormat',1,'MsgComment',{{''}}),'Version',1.2,'general',struct('isFromLib',0)),'OFF',[]}},'GroupId',{{struct('Group',{{'RTICAN'}},'No',2,'Behavior',{{'NAMECHANGE'}},'BlockType',{{'SINK'}},'NameChangeFlag',0),'OFF',[]}},'SFcnRTICANMessage',{{struct('MsgType','RX','SFcnPortType','Scalar','MsgName','PP_Geofence','MsgIdFormat','STD','MsgId',1429,'MsgLength',8,'NumSignals',2,'SampleTime',-1,'Signal',struct('SgnName',{'PP_stop','PP_distance'},'SgnStartBit',{0,16},'SgnLength',{16,16},'SgnType',{'standard','standard'},'ModeValue',{-1,-1},'DataType',{['signed int'],['signed int']},'ByteLayout',{['little endian'],['little endian']},'Factor',{1,1},'Offset',{0,0},'SLDataType',{'SS_DOUBLE','SS_DOUBLE'}),'StatusSelected','yes','TimeSelected','no','DeltaTimeSelected','no','BytePortSelected','no','MessageLengthSelected','no','TriggerPort',struct('Selected','no','TriggerType',0),'UserCoding',struct('Selected','no','InterfaceFile','UserDecodingFile','FcnName','UserDecodeFcn','InportSelected','no','InportWidth',1,'OutportSelected','no','OutportWidth',1),'EnablePortSelected','no','UseRXService','no','BoardType','DS1','BoardNo',1,'ControllerNo',1),'OFF',[]}},'TLCFileName',{{'rtican_rx_message','OFF',[]}})  RTISFcnParameters=struct('SFcnRTICANMessage','struct','TLCFileName','char')  RTIBlockParaDefault=struct('BoardTypeNo',4302,'BoardNo',1,'ChannelNo',1,'Parameters',struct('DataFileSupport',struct('DataFileSelectedMaster',0,'DataFileSelectedLocal',0,'DataFileName','','DataFileDate','','SelectedFile',['<no file selected>']),'Options',struct('StatusSelected',1,'TimeSelected',1,'DeltaTimeSelected',1,'BytePortSelected',0,'MessageLengthSelected',0,'TriggerPort',struct('Selected',0,'TriggerType','rising'),'UserCoding',struct('Selected',0,'InterfaceFile','UserDecodingFile','FcnName','UserDecodeFcn','InportSelected',0,'InportWidth',1,'OutportSelected',0,'OutportWidth',1),'EnablePortSelected',0,'SignalOnPortnameSelected',1,'UseRXService',0),'Message',struct('MsgOnBlocknameSelected',0,'MsgName',['RX Message'],'MsgIdFormat',0,'MsgId',100,'MsgLength',8,'NumSignals',1,'SampleTime',-1,'Signal',struct('SgnName',['RX signal'],'SgnStartBit',0,'SgnLength',8,'SgnType',0,'ModeValue',-1,'DataType',0,'SLDataType','SS_DOUBLE','ByteLayout',0,'Factor',1,'Offset',0,'Min',0,'Max',255,'SgnComment',{{}},'SgnUnit',''),'MsgIdNumFormat',0,'MsgComment',{{''}}),'Version',1.2,'general',struct('isFromLib',1)),'GroupId',struct('Group',{{'RTICAN'}},'No',1,'Behavior',{{'NAMECHANGE'}},'BlockType',{{'SINK'}},'NameChangeFlag',0),'SFcnRTICANMessage',struct('MsgType','RX','MsgName',['RX Message'],'MsgIdFormat','STD','MsgId',100,'MsgLength',8,'NumSignals',1,'SampleTime',-1,'Signal',struct('SgnName',['RX signal'],'SgnStartBit',0,'SgnLength',8,'SgnType','standard','ModeValue',-1,'DataType',['unsigned int'],'ByteLayout',['little endian'],'SLDataType','SS_DOUBLE','Factor',1,'Offset',0),'StatusSelected','yes','TimeSelected','yes','DeltaTimeSelected','yes','BytePortSelected','no','MessageLengthSelected','no','EnablePortSelected','no','UserCoding',struct('Selected','no','InterfaceFile','UserDecodingFile','FcnName','UserDecodeFcn','InportSelected','no','InportWidth',1,'OutportSelected','no','OutportWidth',1),'TriggerPort',struct('Selected','no','TriggerType','rising'),'UseRXService','no','BoardType','DS4302','BoardNo',1,'ControllerNo',1,'SFcnPortType','Scalar'),'TLCFileName','rtican_rx_message')
      settings: AttributesFormatString=Group Id: RTICAN2\n  SourceProductName=dSPACE RTI CAN Blockset
  Radar_Geofence : rtican/RTICAN Receive (RX)   Reserved1=[]  Reserved2=[]  Reserved3=[]  Reserved4=[]  SfcnMessage=[]  Msg_Struct=[]  BoardTypeNo=[]  BoardNo=[]  ChannelNo=[]  Parameters=[]  DialogFcn=[]  UnitName=[]  Revision=[]  UnitValues=[]  DSProperties=struct('RTI',struct('Version',uint32(5),'BlockType',struct('isSLSource',uint8(1),'isSLSink',uint8(1),'isHWSource',uint8(0),'isHWSink',uint8(0),'isSetup',uint8(0),'isInline',uint8(1),'isNonInline',uint8(0),'isInterrupt',uint8(0),'isChannelwise',uint8(0)),'IOBoardType','RTICAN','UnitType','MESSAGE','Identifier','RX','DialogType','MSVC','BlockSet','RTICAN','SlaveProcessor','CAN'))  RTIBlockInterface=struct('OutputPortsWidth',int32([1 1 1 1 1]),'OutputPortsActive',[1 1 1 1 1],'OutputPortsName',{{'GF_TTC','GF_Speed','Nearest_X','Nearest_Y',['RX status']}},'OutputPortsDataType',{{'SS_DOUBLE','SS_DOUBLE','SS_DOUBLE','SS_DOUBLE','SS_DOUBLE'}},'OutputPortsLabel',{{'GF_TTC','GF_Speed','Nearest_X','Nearest_Y',''}},'OutputPortsLabelMode','ON','InputPortsWidth',int32(0),'InputPortsActive',0,'DialogFcn','rtican_message_interface_gui','BlockDisplay',{{'','center'}},'IconTransparency','on','ParameterTunableNames',{{}},'InitLevel',3,'BlockName',struct('Token',{{'Geo_Fence_msg1'}}),'SampleTime',{{-1}},'TriggerPort',{{'none'}},'EnablePort',{{'none'}})  RTIBlockParameters=struct('BoardTypeNo',{{1,'OFF',[]}},'BoardNo',{{1,'ON',[1 16]}},'ChannelNo',{{1,'ON',[1 2]}},'Parameters',{{struct('DataFileSupport',struct('DataFileSelectedMaster',0,'DataFileSelectedLocal',0,'DataFileName',['<no datafile support>|'],'DataFileDate','','SelectedFile',['<no file selected>']),'Options',struct('StatusSelected',1,'TimeSelected',0,'DeltaTimeSelected',0,'BytePortSelected',0,'MessageLengthSelected',0,'TriggerPort',struct('Selected',0,'TriggerType',0),'UserCoding',struct('Selected',0,'InterfaceFile','UserDecodingFile','FcnName','UserDecodeFcn','InportSelected',0,'InportWidth',1,'OutportSelected',0,'OutportWidth',1),'EnablePortSelected',0,'SignalOnPortnameSelected',1,'UseRXService',0),'Message',struct('MsgOnBlocknameSelected',1,'MsgName','Radar_Geofence','MsgIdFormat',0,'MsgId',1426,'MsgLength',8,'NumSignals',4,'SampleTime',-1,'Signal',struct('SgnName',{'GF_TTC','GF_Speed','Nearest_X','Nearest_Y'},'SgnStartBit',{0,16,32,48},'SgnLength',{16,16,16,16},'SgnType',{0,0,0,0},'ModeValue',{-1,-1,-1,-1},'DataType',{1,1,1,1},'ByteLayout',{0,0,0,0},'Factor',{1,1,1,1},'Offset',{0,0,0,0},'SgnComment',{{''},{''},{''},{''}},'SgnUnit',{'','','',''},'Min',{0,0,0,0},'Max',{0,0,0,0},'SLDataType',{'SS_DOUBLE','SS_DOUBLE','SS_DOUBLE','SS_DOUBLE'}),'MsgIdNumFormat',1,'MsgComment',{{''}}),'Version',1.2,'general',struct('isFromLib',0)),'OFF',[]}},'GroupId',{{struct('Group',{{'RTICAN'}},'No',2,'Behavior',{{'NAMECHANGE'}},'BlockType',{{'SINK'}},'NameChangeFlag',0),'OFF',[]}},'SFcnRTICANMessage',{{struct('MsgType','RX','SFcnPortType','Scalar','MsgName','Radar_Geofence','MsgIdFormat','STD','MsgId',1426,'MsgLength',8,'NumSignals',4,'SampleTime',-1,'Signal',struct('SgnName',{'GF_TTC','GF_Speed','Nearest_X','Nearest_Y'},'SgnStartBit',{0,16,32,48},'SgnLength',{16,16,16,16},'SgnType',{'standard','standard','standard','standard'},'ModeValue',{-1,-1,-1,-1},'DataType',{['signed int'],['signed int'],['signed int'],['signed int']},'ByteLayout',{['little endian'],['little endian'],['little endian'],['little endian']},'Factor',{1,1,1,1},'Offset',{0,0,0,0},'SLDataType',{'SS_DOUBLE','SS_DOUBLE','SS_DOUBLE','SS_DOUBLE'}),'StatusSelected','yes','TimeSelected','no','DeltaTimeSelected','no','BytePortSelected','no','MessageLengthSelected','no','TriggerPort',struct('Selected','no','TriggerType',0),'UserCoding',struct('Selected','no','InterfaceFile','UserDecodingFile','FcnName','UserDecodeFcn','InportSelected','no','InportWidth',1,'OutportSelected','no','OutportWidth',1),'EnablePortSelected','no','UseRXService','no','BoardType','DS1','BoardNo',1,'ControllerNo',1),'OFF',[]}},'TLCFileName',{{'rtican_rx_message','OFF',[]}})  RTISFcnParameters=struct('SFcnRTICANMessage','struct','TLCFileName','char')  RTIBlockParaDefault=struct('BoardTypeNo',4302,'BoardNo',1,'ChannelNo',1,'Parameters',struct('DataFileSupport',struct('DataFileSelectedMaster',0,'DataFileSelectedLocal',0,'DataFileName','','DataFileDate','','SelectedFile',['<no file selected>']),'Options',struct('StatusSelected',1,'TimeSelected',1,'DeltaTimeSelected',1,'BytePortSelected',0,'MessageLengthSelected',0,'TriggerPort',struct('Selected',0,'TriggerType','rising'),'UserCoding',struct('Selected',0,'InterfaceFile','UserDecodingFile','FcnName','UserDecodeFcn','InportSelected',0,'InportWidth',1,'OutportSelected',0,'OutportWidth',1),'EnablePortSelected',0,'SignalOnPortnameSelected',1,'UseRXService',0),'Message',struct('MsgOnBlocknameSelected',0,'MsgName',['RX Message'],'MsgIdFormat',0,'MsgId',100,'MsgLength',8,'NumSignals',1,'SampleTime',-1,'Signal',struct('SgnName',['RX signal'],'SgnStartBit',0,'SgnLength',8,'SgnType',0,'ModeValue',-1,'DataType',0,'SLDataType','SS_DOUBLE','ByteLayout',0,'Factor',1,'Offset',0,'Min',0,'Max',255,'SgnComment',{{}},'SgnUnit',''),'MsgIdNumFormat',0,'MsgComment',{{''}}),'Version',1.2,'general',struct('isFromLib',1)),'GroupId',struct('Group',{{'RTICAN'}},'No',1,'Behavior',{{'NAMECHANGE'}},'BlockType',{{'SINK'}},'NameChangeFlag',0),'SFcnRTICANMessage',struct('MsgType','RX','MsgName',['RX Message'],'MsgIdFormat','STD','MsgId',100,'MsgLength',8,'NumSignals',1,'SampleTime',-1,'Signal',struct('SgnName',['RX signal'],'SgnStartBit',0,'SgnLength',8,'SgnType','standard','ModeValue',-1,'DataType',['unsigned int'],'ByteLayout',['little endian'],'SLDataType','SS_DOUBLE','Factor',1,'Offset',0),'StatusSelected','yes','TimeSelected','yes','DeltaTimeSelected','yes','BytePortSelected','no','MessageLengthSelected','no','EnablePortSelected','no','UserCoding',struct('Selected','no','InterfaceFile','UserDecodingFile','FcnName','UserDecodeFcn','InportSelected','no','InportWidth',1,'OutportSelected','no','OutportWidth',1),'TriggerPort',struct('Selected','no','TriggerType','rising'),'UseRXService','no','BoardType','DS4302','BoardNo',1,'ControllerNo',1,'SFcnPortType','Scalar'),'TLCFileName','rtican_rx_message')
      settings: AttributesFormatString=Group Id: RTICAN2\n  SourceProductName=dSPACE RTI CAN Blockset
  Radar_Info : rtican/RTICAN Receive (RX)   Reserved1=[]  Reserved2=[]  Reserved3=[]  Reserved4=[]  SfcnMessage=[]  Msg_Struct=[]  BoardTypeNo=[]  BoardNo=[]  ChannelNo=[]  Parameters=[]  DialogFcn=[]  UnitName=[]  Revision=[]  UnitValues=[]  DSProperties=struct('RTI',struct('Version',uint32(5),'BlockType',struct('isSLSource',uint8(1),'isSLSink',uint8(1),'isHWSource',uint8(0),'isHWSink',uint8(0),'isSetup',uint8(0),'isInline',uint8(1),'isNonInline',uint8(0),'isInterrupt',uint8(0),'isChannelwise',uint8(0)),'IOBoardType','RTICAN','UnitType','MESSAGE','Identifier','RX','DialogType','MSVC','BlockSet','RTICAN','SlaveProcessor','CAN'))  RTIBlockInterface=struct('OutputPortsWidth',int32([1 1 1]),'OutputPortsActive',[1 1 1],'OutputPortsName',{{'Radar_speed','Radar_distance',['RX status']}},'OutputPortsDataType',{{'SS_DOUBLE','SS_DOUBLE','SS_DOUBLE'}},'OutputPortsLabel',{{'Radar_speed','Radar_distance',''}},'OutputPortsLabelMode','ON','InputPortsWidth',int32(0),'InputPortsActive',0,'DialogFcn','rtican_message_interface_gui','BlockDisplay',{{'','center'}},'IconTransparency','on','ParameterTunableNames',{{}},'InitLevel',3,'BlockName',struct('Token',{{'Geo_Fence_Cam1'}}),'SampleTime',{{-1}},'TriggerPort',{{'none'}},'EnablePort',{{'none'}})  RTIBlockParameters=struct('BoardTypeNo',{{1,'OFF',[]}},'BoardNo',{{1,'ON',[1 16]}},'ChannelNo',{{1,'ON',[1 2]}},'Parameters',{{struct('DataFileSupport',struct('DataFileSelectedMaster',0,'DataFileSelectedLocal',0,'DataFileName',['<no datafile support>|'],'DataFileDate','','SelectedFile',['<no file selected>']),'Options',struct('StatusSelected',1,'TimeSelected',0,'DeltaTimeSelected',0,'BytePortSelected',0,'MessageLengthSelected',0,'TriggerPort',struct('Selected',0,'TriggerType',0),'UserCoding',struct('Selected',0,'InterfaceFile','UserDecodingFile','FcnName','UserDecodeFcn','InportSelected',0,'InportWidth',1,'OutportSelected',0,'OutportWidth',1),'EnablePortSelected',0,'SignalOnPortnameSelected',1,'UseRXService',0),'Message',struct('MsgOnBlocknameSelected',1,'MsgName','Geo_Fence_Cam1','MsgIdFormat',0,'MsgId',1586,'MsgLength',8,'NumSignals',2,'SampleTime',-1,'Signal',struct('SgnName',{'Radar_speed','Radar_distance'},'SgnStartBit',{0,32},'SgnLength',{32,32},'SgnType',{0,0},'ModeValue',{-1,-1},'DataType',{1,1},'ByteLayout',{0,0},'Factor',{1,1},'Offset',{0,0},'SgnComment',{{''},{''}},'SgnUnit',{'',''},'Min',{0,0},'Max',{0,0},'SLDataType',{'SS_DOUBLE','SS_DOUBLE'}),'MsgIdNumFormat',1,'MsgComment',{{''}}),'Version',1.2,'general',struct('isFromLib',0)),'OFF',[]}},'GroupId',{{struct('Group',{{'RTICAN'}},'No',2,'Behavior',{{'NAMECHANGE'}},'BlockType',{{'SINK'}},'NameChangeFlag',0),'OFF',[]}},'SFcnRTICANMessage',{{struct('MsgType','RX','SFcnPortType','Scalar','MsgName','Geo_Fence_Cam1','MsgIdFormat','STD','MsgId',1586,'MsgLength',8,'NumSignals',2,'SampleTime',-1,'Signal',struct('SgnName',{'Radar_speed','Radar_distance'},'SgnStartBit',{0,32},'SgnLength',{32,32},'SgnType',{'standard','standard'},'ModeValue',{-1,-1},'DataType',{['signed int'],['signed int']},'ByteLayout',{['little endian'],['little endian']},'Factor',{1,1},'Offset',{0,0},'SLDataType',{'SS_DOUBLE','SS_DOUBLE'}),'StatusSelected','yes','TimeSelected','no','DeltaTimeSelected','no','BytePortSelected','no','MessageLengthSelected','no','TriggerPort',struct('Selected','no','TriggerType',0),'UserCoding',struct('Selected','no','InterfaceFile','UserDecodingFile','FcnName','UserDecodeFcn','InportSelected','no','InportWidth',1,'OutportSelected','no','OutportWidth',1),'EnablePortSelected','no','UseRXService','no','BoardType','DS1','BoardNo',1,'ControllerNo',1),'OFF',[]}},'TLCFileName',{{'rtican_rx_message','OFF',[]}})  RTISFcnParameters=struct('SFcnRTICANMessage','struct','TLCFileName','char')  RTIBlockParaDefault=struct('BoardTypeNo',4302,'BoardNo',1,'ChannelNo',1,'Parameters',struct('DataFileSupport',struct('DataFileSelectedMaster',0,'DataFileSelectedLocal',0,'DataFileName','','DataFileDate','','SelectedFile',['<no file selected>']),'Options',struct('StatusSelected',1,'TimeSelected',1,'DeltaTimeSelected',1,'BytePortSelected',0,'MessageLengthSelected',0,'TriggerPort',struct('Selected',0,'TriggerType','rising'),'UserCoding',struct('Selected',0,'InterfaceFile','UserDecodingFile','FcnName','UserDecodeFcn','InportSelected',0,'InportWidth',1,'OutportSelected',0,'OutportWidth',1),'EnablePortSelected',0,'SignalOnPortnameSelected',1,'UseRXService',0),'Message',struct('MsgOnBlocknameSelected',0,'MsgName',['RX Message'],'MsgIdFormat',0,'MsgId',100,'MsgLength',8,'NumSignals',1,'SampleTime',-1,'Signal',struct('SgnName',['RX signal'],'SgnStartBit',0,'SgnLength',8,'SgnType',0,'ModeValue',-1,'DataType',0,'SLDataType','SS_DOUBLE','ByteLayout',0,'Factor',1,'Offset',0,'Min',0,'Max',255,'SgnComment',{{}},'SgnUnit',''),'MsgIdNumFormat',0,'MsgComment',{{''}}),'Version',1.2,'general',struct('isFromLib',1)),'GroupId',struct('Group',{{'RTICAN'}},'No',1,'Behavior',{{'NAMECHANGE'}},'BlockType',{{'SINK'}},'NameChangeFlag',0),'SFcnRTICANMessage',struct('MsgType','RX','MsgName',['RX Message'],'MsgIdFormat','STD','MsgId',100,'MsgLength',8,'NumSignals',1,'SampleTime',-1,'Signal',struct('SgnName',['RX signal'],'SgnStartBit',0,'SgnLength',8,'SgnType','standard','ModeValue',-1,'DataType',['unsigned int'],'ByteLayout',['little endian'],'SLDataType','SS_DOUBLE','Factor',1,'Offset',0),'StatusSelected','yes','TimeSelected','yes','DeltaTimeSelected','yes','BytePortSelected','no','MessageLengthSelected','no','EnablePortSelected','no','UserCoding',struct('Selected','no','InterfaceFile','UserDecodingFile','FcnName','UserDecodeFcn','InportSelected','no','InportWidth',1,'OutportSelected','no','OutportWidth',1),'TriggerPort',struct('Selected','no','TriggerType','rising'),'UseRXService','no','BoardType','DS4302','BoardNo',1,'ControllerNo',1,'SFcnPortType','Scalar'),'TLCFileName','rtican_rx_message')
      settings: AttributesFormatString=Group Id: RTICAN2\n  SourceProductName=dSPACE RTI CAN Blockset
  Stop_cmd : rtican/RTICAN Receive (RX)   Reserved1=[]  Reserved2=[]  Reserved3=[]  Reserved4=[]  SfcnMessage=[]  Msg_Struct=[]  BoardTypeNo=[]  BoardNo=[]  ChannelNo=[]  Parameters=[]  DialogFcn=[]  UnitName=[]  Revision=[]  UnitValues=[]  DSProperties=struct('RTI',struct('Version',uint32(5),'BlockType',struct('isSLSource',uint8(1),'isSLSink',uint8(1),'isHWSource',uint8(0),'isHWSink',uint8(0),'isSetup',uint8(0),'isInline',uint8(1),'isNonInline',uint8(0),'isInterrupt',uint8(0),'isChannelwise',uint8(0)),'IOBoardType','RTICAN','UnitType','MESSAGE','Identifier','RX','DialogType','MSVC','BlockSet','RTICAN','SlaveProcessor','CAN'))  RTIBlockInterface=struct('OutputPortsWidth',int32([1 1 1 1 1 1 1 1 1]),'OutputPortsActive',[1 1 1 1 1 1 1 1 1],'OutputPortsName',{{'Stop_01','Stop_02','Stop_03','Stop_04','Stop_05','Stop_06','Stop_07','Stop_08',['RX status']}},'OutputPortsDataType',{{'SS_DOUBLE','SS_DOUBLE','SS_DOUBLE','SS_DOUBLE','SS_DOUBLE','SS_DOUBLE','SS_DOUBLE','SS_DOUBLE','SS_DOUBLE'}},'OutputPortsLabel',{{'Stop_01','Stop_02','Stop_03','Stop_04','Stop_05','Stop_06','Stop_07','Stop_08',''}},'OutputPortsLabelMode','ON','InputPortsWidth',int32(0),'InputPortsActive',0,'DialogFcn','rtican_message_interface_gui','BlockDisplay',{{'','center'}},'IconTransparency','on','ParameterTunableNames',{{}},'InitLevel',3,'BlockName',struct('Token',{{'Geo_Fence_msg1'}}),'SampleTime',{{-1}},'TriggerPort',{{'none'}},'EnablePort',{{'none'}})  RTIBlockParameters=struct('BoardTypeNo',{{1,'OFF',[]}},'BoardNo',{{1,'ON',[1 16]}},'ChannelNo',{{1,'ON',[1 2]}},'Parameters',{{struct('DataFileSupport',struct('DataFileSelectedMaster',0,'DataFileSelectedLocal',0,'DataFileName',['<no datafile support>|'],'DataFileDate','','SelectedFile',['<no file selected>']),'Options',struct('StatusSelected',1,'TimeSelected',0,'DeltaTimeSelected',0,'BytePortSelected',0,'MessageLengthSelected',0,'TriggerPort',struct('Selected',0,'TriggerType',0),'UserCoding',struct('Selected',0,'InterfaceFile','UserDecodingFile','FcnName','UserDecodeFcn','InportSelected',0,'InportWidth',1,'OutportSelected',0,'OutportWidth',1),'EnablePortSelected',0,'SignalOnPortnameSelected',1,'UseRXService',0),'Message',struct('MsgOnBlocknameSelected',1,'MsgName','Stop_cmd','MsgIdFormat',0,'MsgId',85,'MsgLength',8,'NumSignals',8,'SampleTime',-1,'Signal',struct('SgnName',{'Stop_01','Stop_02','Stop_03','Stop_04','Stop_05','Stop_06','Stop_07','Stop_08'},'SgnStartBit',{0,8,16,24,32,40,48,56},'SgnLength',{8,8,8,8,8,8,8,8},'SgnType',{0,0,0,0,0,0,0,0},'ModeValue',{-1,-1,-1,-1,-1,-1,-1,-1},'DataType',{0,0,0,0,0,0,0,0},'ByteLayout',{0,0,0,0,0,0,0,0},'Factor',{1,1,1,1,1,1,1,1},'Offset',{0,0,0,0,0,0,0,0},'SgnComment',{{''},{''},{''},{''},{''},{''},{''},{''}},'SgnUnit',{'','','','','','','',''},'Min',{0,0,0,0,0,0,0,0},'Max',{0,0,0,0,0,0,0,0},'SLDataType',{'SS_DOUBLE','SS_DOUBLE','SS_DOUBLE','SS_DOUBLE','SS_DOUBLE','SS_DOUBLE','SS_DOUBLE','SS_DOUBLE'}),'MsgIdNumFormat',1,'MsgComment',{{''}}),'Version',1.2,'general',struct('isFromLib',0)),'OFF',[]}},'GroupId',{{struct('Group',{{'RTICAN'}},'No',2,'Behavior',{{'NAMECHANGE'}},'BlockType',{{'SINK'}},'NameChangeFlag',0),'OFF',[]}},'SFcnRTICANMessage',{{struct('MsgType','RX','SFcnPortType','Scalar','MsgName','Stop_cmd','MsgIdFormat','STD','MsgId',85,'MsgLength',8,'NumSignals',8,'SampleTime',-1,'Signal',struct('SgnName',{'Stop_01','Stop_02','Stop_03','Stop_04','Stop_05','Stop_06','Stop_07','Stop_08'},'SgnStartBit',{0,8,16,24,32,40,48,56},'SgnLength',{8,8,8,8,8,8,8,8},'SgnType',{'standard','standard','standard','standard','standard','standard','standard','standard'},'ModeValue',{-1,-1,-1,-1,-1,-1,-1,-1},'DataType',{['unsigned int'],['unsigned int'],['unsigned int'],['unsigned int'],['unsigned int'],['unsigned int'],['unsigned int'],['unsigned int']},'ByteLayout',{['little endian'],['little endian'],['little endian'],['little endian'],['little endian'],['little endian'],['little endian'],['little endian']},'Factor',{1,1,1,1,1,1,1,1},'Offset',{0,0,0,0,0,0,0,0},'SLDataType',{'SS_DOUBLE','SS_DOUBLE','SS_DOUBLE','SS_DOUBLE','SS_DOUBLE','SS_DOUBLE','SS_DOUBLE','SS_DOUBLE'}),'StatusSelected','yes','TimeSelected','no','DeltaTimeSelected','no','BytePortSelected','no','MessageLengthSelected','no','TriggerPort',struct('Selected','no','TriggerType',0),'UserCoding',struct('Selected','no','InterfaceFile','UserDecodingFile','FcnName','UserDecodeFcn','InportSelected','no','InportWidth',1,'OutportSelected','no','OutportWidth',1),'EnablePortSelected','no','UseRXService','no','BoardType','DS1','BoardNo',1,'ControllerNo',1),'OFF',[]}},'TLCFileName',{{'rtican_rx_message','OFF',[]}})  RTISFcnParameters=struct('SFcnRTICANMessage','struct','TLCFileName','char')  RTIBlockParaDefault=struct('BoardTypeNo',4302,'BoardNo',1,'ChannelNo',1,'Parameters',struct('DataFileSupport',struct('DataFileSelectedMaster',0,'DataFileSelectedLocal',0,'DataFileName','','DataFileDate','','SelectedFile',['<no file selected>']),'Options',struct('StatusSelected',1,'TimeSelected',1,'DeltaTimeSelected',1,'BytePortSelected',0,'MessageLengthSelected',0,'TriggerPort',struct('Selected',0,'TriggerType','rising'),'UserCoding',struct('Selected',0,'InterfaceFile','UserDecodingFile','FcnName','UserDecodeFcn','InportSelected',0,'InportWidth',1,'OutportSelected',0,'OutportWidth',1),'EnablePortSelected',0,'SignalOnPortnameSelected',1,'UseRXService',0),'Message',struct('MsgOnBlocknameSelected',0,'MsgName',['RX Message'],'MsgIdFormat',0,'MsgId',100,'MsgLength',8,'NumSignals',1,'SampleTime',-1,'Signal',struct('SgnName',['RX signal'],'SgnStartBit',0,'SgnLength',8,'SgnType',0,'ModeValue',-1,'DataType',0,'SLDataType','SS_DOUBLE','ByteLayout',0,'Factor',1,'Offset',0,'Min',0,'Max',255,'SgnComment',{{}},'SgnUnit',''),'MsgIdNumFormat',0,'MsgComment',{{''}}),'Version',1.2,'general',struct('isFromLib',1)),'GroupId',struct('Group',{{'RTICAN'}},'No',1,'Behavior',{{'NAMECHANGE'}},'BlockType',{{'SINK'}},'NameChangeFlag',0),'SFcnRTICANMessage',struct('MsgType','RX','MsgName',['RX Message'],'MsgIdFormat','STD','MsgId',100,'MsgLength',8,'NumSignals',1,'SampleTime',-1,'Signal',struct('SgnName',['RX signal'],'SgnStartBit',0,'SgnLength',8,'SgnType','standard','ModeValue',-1,'DataType',['unsigned int'],'ByteLayout',['little endian'],'SLDataType','SS_DOUBLE','Factor',1,'Offset',0),'StatusSelected','yes','TimeSelected','yes','DeltaTimeSelected','yes','BytePortSelected','no','MessageLengthSelected','no','EnablePortSelected','no','UserCoding',struct('Selected','no','InterfaceFile','UserDecodingFile','FcnName','UserDecodeFcn','InportSelected','no','InportWidth',1,'OutportSelected','no','OutportWidth',1),'TriggerPort',struct('Selected','no','TriggerType','rising'),'UseRXService','no','BoardType','DS4302','BoardNo',1,'ControllerNo',1,'SFcnPortType','Scalar'),'TLCFileName','rtican_rx_message')
      settings: AttributesFormatString=Group Id: RTICAN2\n  SourceProductName=dSPACE RTI CAN Blockset
  Switch : Switch  Criteria=u2 > Threshold  Threshold=100
  Switch4 : Switch  Criteria=u2 > Threshold
  System_ready : rtican/RTICAN Receive (RX)   Reserved1=[]  Reserved2=[]  Reserved3=[]  Reserved4=[]  SfcnMessage=[]  Msg_Struct=[]  BoardTypeNo=[]  BoardNo=[]  ChannelNo=[]  Parameters=[]  DialogFcn=[]  UnitName=[]  Revision=[]  UnitValues=[]  DSProperties=struct('RTI',struct('Version',uint32(5),'BlockType',struct('isSLSource',uint8(1),'isSLSink',uint8(1),'isHWSource',uint8(0),'isHWSink',uint8(0),'isSetup',uint8(0),'isInline',uint8(1),'isNonInline',uint8(0),'isInterrupt',uint8(0),'isChannelwise',uint8(0)),'IOBoardType','RTICAN','UnitType','MESSAGE','Identifier','RX','DialogType','MSVC','BlockSet','RTICAN','SlaveProcessor','CAN'))  RTIBlockInterface=struct('OutputPortsWidth',int32([1 1]),'OutputPortsActive',[1 1],'OutputPortsName',{{'System_ready',['RX status']}},'OutputPortsDataType',{{'SS_DOUBLE','SS_DOUBLE'}},'OutputPortsLabel',{{'System_ready',''}},'OutputPortsLabelMode','ON','InputPortsWidth',int32(0),'InputPortsActive',0,'DialogFcn','rtican_message_interface_gui','BlockDisplay',{{'','center'}},'IconTransparency','on','ParameterTunableNames',{{}},'InitLevel',3,'BlockName',struct('Token',{{'System_ready'}}),'SampleTime',{{-1}},'TriggerPort',{{'none'}},'EnablePort',{{'none'}})  RTIBlockParameters=struct('BoardTypeNo',{{1,'OFF',[]}},'BoardNo',{{1,'ON',[1 16]}},'ChannelNo',{{1,'ON',[1 2]}},'Parameters',{{struct('DataFileSupport',struct('DataFileSelectedMaster',0,'DataFileSelectedLocal',0,'DataFileName',['<no datafile support>|'],'DataFileDate','','SelectedFile',['<no file selected>']),'Options',struct('StatusSelected',1,'TimeSelected',0,'DeltaTimeSelected',0,'BytePortSelected',0,'MessageLengthSelected',0,'TriggerPort',struct('Selected',0,'TriggerType',0),'UserCoding',struct('Selected',0,'InterfaceFile','UserDecodingFile','FcnName','UserDecodeFcn','InportSelected',0,'InportWidth',1,'OutportSelected',0,'OutportWidth',1),'EnablePortSelected',0,'SignalOnPortnameSelected',1,'UseRXService',0),'Message',struct('MsgOnBlocknameSelected',1,'MsgName','System_ready','MsgIdFormat',0,'MsgId',81,'MsgLength',8,'NumSignals',1,'SampleTime',-1,'Signal',struct('SgnName','System_ready','SgnStartBit',0,'SgnLength',16,'SgnType',0,'ModeValue',-1,'DataType',0,'ByteLayout',0,'Factor',1,'Offset',0,'SgnComment',{{''}},'SgnUnit','','Min',0,'Max',0,'SLDataType','SS_DOUBLE'),'MsgIdNumFormat',1,'MsgComment',{{''}}),'Version',1.2,'general',struct('isFromLib',0)),'OFF',[]}},'GroupId',{{struct('Group',{{'RTICAN'}},'No',2,'Behavior',{{'NAMECHANGE'}},'BlockType',{{'SINK'}},'NameChangeFlag',0),'OFF',[]}},'SFcnRTICANMessage',{{struct('MsgType','RX','SFcnPortType','Scalar','MsgName','System_ready','MsgIdFormat','STD','MsgId',81,'MsgLength',8,'NumSignals',1,'SampleTime',-1,'Signal',struct('SgnName','System_ready','SgnStartBit',0,'SgnLength',16,'SgnType','standard','ModeValue',-1,'DataType',['unsigned int'],'ByteLayout',['little endian'],'Factor',1,'Offset',0,'SLDataType','SS_DOUBLE'),'StatusSelected','yes','TimeSelected','no','DeltaTimeSelected','no','BytePortSelected','no','MessageLengthSelected','no','TriggerPort',struct('Selected','no','TriggerType',0),'UserCoding',struct('Selected','no','InterfaceFile','UserDecodingFile','FcnName','UserDecodeFcn','InportSelected','no','InportWidth',1,'OutportSelected','no','OutportWidth',1),'EnablePortSelected','no','UseRXService','no','BoardType','DS1','BoardNo',1,'ControllerNo',1),'OFF',[]}},'TLCFileName',{{'rtican_rx_message','OFF',[]}})  RTISFcnParameters=struct('SFcnRTICANMessage','struct','TLCFileName','char')  RTIBlockParaDefault=struct('BoardTypeNo',4302,'BoardNo',1,'ChannelNo',1,'Parameters',struct('DataFileSupport',struct('DataFileSelectedMaster',0,'DataFileSelectedLocal',0,'DataFileName','','DataFileDate','','SelectedFile',['<no file selected>']),'Options',struct('StatusSelected',1,'TimeSelected',1,'DeltaTimeSelected',1,'BytePortSelected',0,'MessageLengthSelected',0,'TriggerPort',struct('Selected',0,'TriggerType','rising'),'UserCoding',struct('Selected',0,'InterfaceFile','UserDecodingFile','FcnName','UserDecodeFcn','InportSelected',0,'InportWidth',1,'OutportSelected',0,'OutportWidth',1),'EnablePortSelected',0,'SignalOnPortnameSelected',1,'UseRXService',0),'Message',struct('MsgOnBlocknameSelected',0,'MsgName',['RX Message'],'MsgIdFormat',0,'MsgId',100,'MsgLength',8,'NumSignals',1,'SampleTime',-1,'Signal',struct('SgnName',['RX signal'],'SgnStartBit',0,'SgnLength',8,'SgnType',0,'ModeValue',-1,'DataType',0,'SLDataType','SS_DOUBLE','ByteLayout',0,'Factor',1,'Offset',0,'Min',0,'Max',255,'SgnComment',{{}},'SgnUnit',''),'MsgIdNumFormat',0,'MsgComment',{{''}}),'Version',1.2,'general',struct('isFromLib',1)),'GroupId',struct('Group',{{'RTICAN'}},'No',1,'Behavior',{{'NAMECHANGE'}},'BlockType',{{'SINK'}},'NameChangeFlag',0),'SFcnRTICANMessage',struct('MsgType','RX','MsgName',['RX Message'],'MsgIdFormat','STD','MsgId',100,'MsgLength',8,'NumSignals',1,'SampleTime',-1,'Signal',struct('SgnName',['RX signal'],'SgnStartBit',0,'SgnLength',8,'SgnType','standard','ModeValue',-1,'DataType',['unsigned int'],'ByteLayout',['little endian'],'SLDataType','SS_DOUBLE','Factor',1,'Offset',0),'StatusSelected','yes','TimeSelected','yes','DeltaTimeSelected','yes','BytePortSelected','no','MessageLengthSelected','no','EnablePortSelected','no','UserCoding',struct('Selected','no','InterfaceFile','UserDecodingFile','FcnName','UserDecodeFcn','InportSelected','no','InportWidth',1,'OutportSelected','no','OutportWidth',1),'TriggerPort',struct('Selected','no','TriggerType','rising'),'UseRXService','no','BoardType','DS4302','BoardNo',1,'ControllerNo',1,'SFcnPortType','Scalar'),'TLCFileName','rtican_rx_message')
      settings: AttributesFormatString=Group Id: RTICAN2\n  SourceProductName=dSPACE RTI CAN Blockset
  TouchP_start : rtican/RTICAN Receive (RX)   Reserved1=[]  Reserved2=[]  Reserved3=[]  Reserved4=[]  SfcnMessage=[]  Msg_Struct=[]  BoardTypeNo=[]  BoardNo=[]  ChannelNo=[]  Parameters=[]  DialogFcn=[]  UnitName=[]  Revision=[]  UnitValues=[]  DSProperties=struct('RTI',struct('Version',uint32(5),'BlockType',struct('isSLSource',uint8(1),'isSLSink',uint8(1),'isHWSource',uint8(0),'isHWSink',uint8(0),'isSetup',uint8(0),'isInline',uint8(1),'isNonInline',uint8(0),'isInterrupt',uint8(0),'isChannelwise',uint8(0)),'IOBoardType','RTICAN','UnitType','MESSAGE','Identifier','RX','DialogType','MSVC','BlockSet','RTICAN','SlaveProcessor','CAN'))  RTIBlockInterface=struct('OutputPortsWidth',int32([1 1]),'OutputPortsActive',[1 1],'OutputPortsName',{{'TouchP_start',['RX status']}},'OutputPortsDataType',{{'SS_DOUBLE','SS_DOUBLE'}},'OutputPortsLabel',{{'TouchP_start',''}},'OutputPortsLabelMode','ON','InputPortsWidth',int32(0),'InputPortsActive',0,'DialogFcn','rtican_message_interface_gui','BlockDisplay',{{'','center'}},'IconTransparency','on','ParameterTunableNames',{{}},'InitLevel',3,'BlockName',struct('Token',{{'Geo_Fence_msg1'}}),'SampleTime',{{-1}},'TriggerPort',{{'none'}},'EnablePort',{{'none'}})  RTIBlockParameters=struct('BoardTypeNo',{{1,'OFF',[]}},'BoardNo',{{1,'ON',[1 16]}},'ChannelNo',{{1,'ON',[1 2]}},'Parameters',{{struct('DataFileSupport',struct('DataFileSelectedMaster',0,'DataFileSelectedLocal',0,'DataFileName',['<no datafile support>|'],'DataFileDate','','SelectedFile',['<no file selected>']),'Options',struct('StatusSelected',1,'TimeSelected',0,'DeltaTimeSelected',0,'BytePortSelected',0,'MessageLengthSelected',0,'TriggerPort',struct('Selected',0,'TriggerType',0),'UserCoding',struct('Selected',0,'InterfaceFile','UserDecodingFile','FcnName','UserDecodeFcn','InportSelected',0,'InportWidth',1,'OutportSelected',0,'OutportWidth',1),'EnablePortSelected',0,'SignalOnPortnameSelected',1,'UseRXService',0),'Message',struct('MsgOnBlocknameSelected',1,'MsgName','TouchP_start','MsgIdFormat',0,'MsgId',80,'MsgLength',8,'NumSignals',1,'SampleTime',-1,'Signal',struct('SgnName','TouchP_start','SgnStartBit',0,'SgnLength',16,'SgnType',0,'ModeValue',-1,'DataType',0,'ByteLayout',0,'Factor',1,'Offset',0,'SgnComment',{{''}},'SgnUnit','','Min',0,'Max',0,'SLDataType','SS_DOUBLE'),'MsgIdNumFormat',1,'MsgComment',{{''}}),'Version',1.2,'general',struct('isFromLib',0)),'OFF',[]}},'GroupId',{{struct('Group',{{'RTICAN'}},'No',2,'Behavior',{{'NAMECHANGE'}},'BlockType',{{'SINK'}},'NameChangeFlag',0),'OFF',[]}},'SFcnRTICANMessage',{{struct('MsgType','RX','SFcnPortType','Scalar','MsgName','TouchP_start','MsgIdFormat','STD','MsgId',80,'MsgLength',8,'NumSignals',1,'SampleTime',-1,'Signal',struct('SgnName','TouchP_start','SgnStartBit',0,'SgnLength',16,'SgnType','standard','ModeValue',-1,'DataType',['unsigned int'],'ByteLayout',['little endian'],'Factor',1,'Offset',0,'SLDataType','SS_DOUBLE'),'StatusSelected','yes','TimeSelected','no','DeltaTimeSelected','no','BytePortSelected','no','MessageLengthSelected','no','TriggerPort',struct('Selected','no','TriggerType',0),'UserCoding',struct('Selected','no','InterfaceFile','UserDecodingFile','FcnName','UserDecodeFcn','InportSelected','no','InportWidth',1,'OutportSelected','no','OutportWidth',1),'EnablePortSelected','no','UseRXService','no','BoardType','DS1','BoardNo',1,'ControllerNo',1),'OFF',[]}},'TLCFileName',{{'rtican_rx_message','OFF',[]}})  RTISFcnParameters=struct('SFcnRTICANMessage','struct','TLCFileName','char')  RTIBlockParaDefault=struct('BoardTypeNo',4302,'BoardNo',1,'ChannelNo',1,'Parameters',struct('DataFileSupport',struct('DataFileSelectedMaster',0,'DataFileSelectedLocal',0,'DataFileName','','DataFileDate','','SelectedFile',['<no file selected>']),'Options',struct('StatusSelected',1,'TimeSelected',1,'DeltaTimeSelected',1,'BytePortSelected',0,'MessageLengthSelected',0,'TriggerPort',struct('Selected',0,'TriggerType','rising'),'UserCoding',struct('Selected',0,'InterfaceFile','UserDecodingFile','FcnName','UserDecodeFcn','InportSelected',0,'InportWidth',1,'OutportSelected',0,'OutportWidth',1),'EnablePortSelected',0,'SignalOnPortnameSelected',1,'UseRXService',0),'Message',struct('MsgOnBlocknameSelected',0,'MsgName',['RX Message'],'MsgIdFormat',0,'MsgId',100,'MsgLength',8,'NumSignals',1,'SampleTime',-1,'Signal',struct('SgnName',['RX signal'],'SgnStartBit',0,'SgnLength',8,'SgnType',0,'ModeValue',-1,'DataType',0,'SLDataType','SS_DOUBLE','ByteLayout',0,'Factor',1,'Offset',0,'Min',0,'Max',255,'SgnComment',{{}},'SgnUnit',''),'MsgIdNumFormat',0,'MsgComment',{{''}}),'Version',1.2,'general',struct('isFromLib',1)),'GroupId',struct('Group',{{'RTICAN'}},'No',1,'Behavior',{{'NAMECHANGE'}},'BlockType',{{'SINK'}},'NameChangeFlag',0),'SFcnRTICANMessage',struct('MsgType','RX','MsgName',['RX Message'],'MsgIdFormat','STD','MsgId',100,'MsgLength',8,'NumSignals',1,'SampleTime',-1,'Signal',struct('SgnName',['RX signal'],'SgnStartBit',0,'SgnLength',8,'SgnType','standard','ModeValue',-1,'DataType',['unsigned int'],'ByteLayout',['little endian'],'SLDataType','SS_DOUBLE','Factor',1,'Offset',0),'StatusSelected','yes','TimeSelected','yes','DeltaTimeSelected','yes','BytePortSelected','no','MessageLengthSelected','no','EnablePortSelected','no','UserCoding',struct('Selected','no','InterfaceFile','UserDecodingFile','FcnName','UserDecodeFcn','InportSelected','no','InportWidth',1,'OutportSelected','no','OutportWidth',1),'TriggerPort',struct('Selected','no','TriggerType','rising'),'UseRXService','no','BoardType','DS4302','BoardNo',1,'ControllerNo',1,'SFcnPortType','Scalar'),'TLCFileName','rtican_rx_message')
      settings: AttributesFormatString=Group Id: RTICAN2\n  SourceProductName=dSPACE RTI CAN Blockset
  Traffic_light : rtican/RTICAN Receive (RX)   Reserved1=[]  Reserved2=[]  Reserved3=[]  Reserved4=[]  SfcnMessage=[]  Msg_Struct=[]  BoardTypeNo=[]  BoardNo=[]  ChannelNo=[]  Parameters=[]  DialogFcn=[]  UnitName=[]  Revision=[]  UnitValues=[]  DSProperties=struct('RTI',struct('Version',uint32(5),'BlockType',struct('isSLSource',uint8(1),'isSLSink',uint8(1),'isHWSource',uint8(0),'isHWSink',uint8(0),'isSetup',uint8(0),'isInline',uint8(1),'isNonInline',uint8(0),'isInterrupt',uint8(0),'isChannelwise',uint8(0)),'IOBoardType','RTICAN','UnitType','MESSAGE','Identifier','RX','DialogType','MSVC','BlockSet','RTICAN','SlaveProcessor','CAN'))  RTIBlockInterface=struct('OutputPortsWidth',int32([1 1 1]),'OutputPortsActive',[1 1 1],'OutputPortsName',{{'color_light','direction',['RX status']}},'OutputPortsDataType',{{'SS_DOUBLE','SS_DOUBLE','SS_DOUBLE'}},'OutputPortsLabel',{{'color_light','direction',''}},'OutputPortsLabelMode','ON','InputPortsWidth',int32(0),'InputPortsActive',0,'DialogFcn','rtican_message_interface_gui','BlockDisplay',{{'','center'}},'IconTransparency','on','ParameterTunableNames',{{}},'InitLevel',3,'BlockName',struct('Token',{{'Traffic_light'}}),'SampleTime',{{-1}},'TriggerPort',{{'none'}},'EnablePort',{{'none'}})  RTIBlockParameters=struct('BoardTypeNo',{{1,'OFF',[]}},'BoardNo',{{1,'ON',[1 16]}},'ChannelNo',{{1,'ON',[1 2]}},'Parameters',{{struct('DataFileSupport',struct('DataFileSelectedMaster',0,'DataFileSelectedLocal',0,'DataFileName',['<no datafile support>|'],'DataFileDate','','SelectedFile',['<no file selected>']),'Options',struct('StatusSelected',1,'TimeSelected',0,'DeltaTimeSelected',0,'BytePortSelected',0,'MessageLengthSelected',0,'TriggerPort',struct('Selected',0,'TriggerType',0),'UserCoding',struct('Selected',0,'InterfaceFile','UserDecodingFile','FcnName','UserDecodeFcn','InportSelected',0,'InportWidth',1,'OutportSelected',0,'OutportWidth',1),'EnablePortSelected',0,'SignalOnPortnameSelected',1,'UseRXService',0),'Message',struct('MsgOnBlocknameSelected',1,'MsgName','Traffic_light','MsgIdFormat',0,'MsgId',97,'MsgLength',8,'NumSignals',2,'SampleTime',-1,'Signal',struct('SgnName',{'color_light','direction'},'SgnStartBit',{0,16},'SgnLength',{16,16},'SgnType',{0,0},'ModeValue',{-1,-1},'DataType',{0,0},'ByteLayout',{0,0},'Factor',{1,1},'Offset',{0,0},'SgnComment',{{''},{''}},'SgnUnit',{'',''},'Min',{0,0},'Max',{0,0},'SLDataType',{'SS_DOUBLE','SS_DOUBLE'}),'MsgIdNumFormat',1,'MsgComment',{{''}}),'Version',1.2,'general',struct('isFromLib',0)),'OFF',[]}},'GroupId',{{struct('Group',{{'RTICAN'}},'No',2,'Behavior',{{'NAMECHANGE'}},'BlockType',{{'SINK'}},'NameChangeFlag',0),'OFF',[]}},'SFcnRTICANMessage',{{struct('MsgType','RX','SFcnPortType','Scalar','MsgName','Traffic_light','MsgIdFormat','STD','MsgId',97,'MsgLength',8,'NumSignals',2,'SampleTime',-1,'Signal',struct('SgnName',{'color_light','direction'},'SgnStartBit',{0,16},'SgnLength',{16,16},'SgnType',{'standard','standard'},'ModeValue',{-1,-1},'DataType',{['unsigned int'],['unsigned int']},'ByteLayout',{['little endian'],['little endian']},'Factor',{1,1},'Offset',{0,0},'SLDataType',{'SS_DOUBLE','SS_DOUBLE'}),'StatusSelected','yes','TimeSelected','no','DeltaTimeSelected','no','BytePortSelected','no','MessageLengthSelected','no','TriggerPort',struct('Selected','no','TriggerType',0),'UserCoding',struct('Selected','no','InterfaceFile','UserDecodingFile','FcnName','UserDecodeFcn','InportSelected','no','InportWidth',1,'OutportSelected','no','OutportWidth',1),'EnablePortSelected','no','UseRXService','no','BoardType','DS1','BoardNo',1,'ControllerNo',1),'OFF',[]}},'TLCFileName',{{'rtican_rx_message','OFF',[]}})  RTISFcnParameters=struct('SFcnRTICANMessage','struct','TLCFileName','char')  RTIBlockParaDefault=struct('BoardTypeNo',4302,'BoardNo',1,'ChannelNo',1,'Parameters',struct('DataFileSupport',struct('DataFileSelectedMaster',0,'DataFileSelectedLocal',0,'DataFileName','','DataFileDate','','SelectedFile',['<no file selected>']),'Options',struct('StatusSelected',1,'TimeSelected',1,'DeltaTimeSelected',1,'BytePortSelected',0,'MessageLengthSelected',0,'TriggerPort',struct('Selected',0,'TriggerType','rising'),'UserCoding',struct('Selected',0,'InterfaceFile','UserDecodingFile','FcnName','UserDecodeFcn','InportSelected',0,'InportWidth',1,'OutportSelected',0,'OutportWidth',1),'EnablePortSelected',0,'SignalOnPortnameSelected',1,'UseRXService',0),'Message',struct('MsgOnBlocknameSelected',0,'MsgName',['RX Message'],'MsgIdFormat',0,'MsgId',100,'MsgLength',8,'NumSignals',1,'SampleTime',-1,'Signal',struct('SgnName',['RX signal'],'SgnStartBit',0,'SgnLength',8,'SgnType',0,'ModeValue',-1,'DataType',0,'SLDataType','SS_DOUBLE','ByteLayout',0,'Factor',1,'Offset',0,'Min',0,'Max',255,'SgnComment',{{}},'SgnUnit',''),'MsgIdNumFormat',0,'MsgComment',{{''}}),'Version',1.2,'general',struct('isFromLib',1)),'GroupId',struct('Group',{{'RTICAN'}},'No',1,'Behavior',{{'NAMECHANGE'}},'BlockType',{{'SINK'}},'NameChangeFlag',0),'SFcnRTICANMessage',struct('MsgType','RX','MsgName',['RX Message'],'MsgIdFormat','STD','MsgId',100,'MsgLength',8,'NumSignals',1,'SampleTime',-1,'Signal',struct('SgnName',['RX signal'],'SgnStartBit',0,'SgnLength',8,'SgnType','standard','ModeValue',-1,'DataType',['unsigned int'],'ByteLayout',['little endian'],'SLDataType','SS_DOUBLE','Factor',1,'Offset',0),'StatusSelected','yes','TimeSelected','yes','DeltaTimeSelected','yes','BytePortSelected','no','MessageLengthSelected','no','EnablePortSelected','no','UserCoding',struct('Selected','no','InterfaceFile','UserDecodingFile','FcnName','UserDecodeFcn','InportSelected','no','InportWidth',1,'OutportSelected','no','OutportWidth',1),'TriggerPort',struct('Selected','no','TriggerType','rising'),'UseRXService','no','BoardType','DS4302','BoardNo',1,'ControllerNo',1,'SFcnPortType','Scalar'),'TLCFileName','rtican_rx_message')
      settings: AttributesFormatString=Group Id: RTICAN2\n  SourceProductName=dSPACE RTI CAN Blockset
  Unit Delay : UnitDelay  SampleTime=-1
  Unit Delay1 : UnitDelay  SampleTime=-1
  Unit Delay2 : UnitDelay  InitialCondition=300  SampleTime=-1
  "[Disp] BBGF_Distance" : Display
  "[Disp] BBGF_NearestX" : Display
  "[Disp] BBGF_NearestY" : Display
  "[Disp] BBGF_Speed" : Display
  "[Disp] DeviatePath_Distance" : Display
  "[Disp] DeviatePath_Distance_raw" : Display
  "[Disp] DeviatePath_NearestX" : Display
  "[Disp] DeviatePath_NearestY" : Display
  "[Disp] DeviatePath_Speed" : Display
  "[Disp] GF_Distance" : Display
  "[Disp] GF_Speed" : Display
  "[Disp] PCGF_Distance" : Display
  "[Disp] PCGF_Distance_raw" : Display
  "[Disp] PCGF_NearestX" : Display
  "[Disp] PCGF_NearestY" : Display
  "[Disp] PCGF_Speed" : Display
  "[Disp] PPGF_Stop" : Display
  "[Disp] PPGF_distance" : Display
  "[Disp] RDGF_Distance" : Display
  "[Disp] RDGF_NearestX" : Display
  "[Disp] RDGF_NearestY" : Display
  "[Disp] RDGF_Speed" : Display
  "[Disp] RX_BBox_Geofence" : Display
  "[Disp] RX_BBox_Geofence1" : Display
  "[Disp] RX_PCloud_Geofence" : Display
  "[Disp] RX_PCloud_Geofence1" : Display
  "[Disp] RX_PP_Geofence" : Display
  "[Disp] RX_overtake_over" : Display
  "[Disp] Radar_RX" : Display
  "[Disp] Radar_distance" : Display
  "[Disp] Radar_speed" : Display
  "[Disp] Radar_update_gap" : Display
  [Disp] Stop_cmd{,1..8} (9 alike) : Display
  "[Disp] Stop_cmd_RX" : Display
  "[Disp] System_ready" : Display
  "[Disp] TouchP_start" : Display
  "[Disp] TouchP_start_RX" : Display
  "[Disp] color_light" : Display
  "[Disp] direction_light" : Display
  "[Disp] overtake_over" : Display
  "[Para]DV_enable" : Constant  Value=0
  "[Para]GF_Dis_switch" : Constant  Value=2
  "[Para]GF_Spd_switch" : Constant
  overtake_over : rtican/RTICAN Receive (RX)   Reserved1=[]  Reserved2=[]  Reserved3=[]  Reserved4=[]  SfcnMessage=[]  Msg_Struct=[]  BoardTypeNo=[]  BoardNo=[]  ChannelNo=[]  Parameters=[]  DialogFcn=[]  UnitName=[]  Revision=[]  UnitValues=[]  DSProperties=struct('RTI',struct('Version',uint32(5),'BlockType',struct('isSLSource',uint8(1),'isSLSink',uint8(1),'isHWSource',uint8(0),'isHWSink',uint8(0),'isSetup',uint8(0),'isInline',uint8(1),'isNonInline',uint8(0),'isInterrupt',uint8(0),'isChannelwise',uint8(0)),'IOBoardType','RTICAN','UnitType','MESSAGE','Identifier','RX','DialogType','MSVC','BlockSet','RTICAN','SlaveProcessor','CAN'))  RTIBlockInterface=struct('OutputPortsWidth',int32([1 1]),'OutputPortsActive',[1 1],'OutputPortsName',{{'overtake_over',['RX status']}},'OutputPortsDataType',{{'SS_DOUBLE','SS_DOUBLE'}},'OutputPortsLabel',{{'overtake_over',''}},'OutputPortsLabelMode','ON','InputPortsWidth',int32(0),'InputPortsActive',0,'DialogFcn','rtican_message_interface_gui','BlockDisplay',{{'','center'}},'IconTransparency','on','ParameterTunableNames',{{}},'InitLevel',3,'BlockName',struct('Token',{{'overtake_over'}}),'SampleTime',{{-1}},'TriggerPort',{{'none'}},'EnablePort',{{'none'}})  RTIBlockParameters=struct('BoardTypeNo',{{1,'OFF',[]}},'BoardNo',{{1,'ON',[1 16]}},'ChannelNo',{{1,'ON',[1 2]}},'Parameters',{{struct('DataFileSupport',struct('DataFileSelectedMaster',0,'DataFileSelectedLocal',0,'DataFileName',['<no datafile support>|'],'DataFileDate','','SelectedFile',['<no file selected>']),'Options',struct('StatusSelected',1,'TimeSelected',0,'DeltaTimeSelected',0,'BytePortSelected',0,'MessageLengthSelected',0,'TriggerPort',struct('Selected',0,'TriggerType',0),'UserCoding',struct('Selected',0,'InterfaceFile','UserDecodingFile','FcnName','UserDecodeFcn','InportSelected',0,'InportWidth',1,'OutportSelected',0,'OutportWidth',1),'EnablePortSelected',0,'SignalOnPortnameSelected',1,'UseRXService',0),'Message',struct('MsgOnBlocknameSelected',1,'MsgName','overtake_over','MsgIdFormat',0,'MsgId',1433,'MsgLength',8,'NumSignals',1,'SampleTime',-1,'Signal',struct('SgnName','overtake_over','SgnStartBit',0,'SgnLength',16,'SgnType',0,'ModeValue',-1,'DataType',1,'ByteLayout',0,'Factor',1,'Offset',0,'SgnComment',{{''}},'SgnUnit','','Min',0,'Max',0,'SLDataType','SS_DOUBLE'),'MsgIdNumFormat',1,'MsgComment',{{''}}),'Version',1.2,'general',struct('isFromLib',0)),'OFF',[]}},'GroupId',{{struct('Group',{{'RTICAN'}},'No',2,'Behavior',{{'NAMECHANGE'}},'BlockType',{{'SINK'}},'NameChangeFlag',0),'OFF',[]}},'SFcnRTICANMessage',{{struct('MsgType','RX','SFcnPortType','Scalar','MsgName','overtake_over','MsgIdFormat','STD','MsgId',1433,'MsgLength',8,'NumSignals',1,'SampleTime',-1,'Signal',struct('SgnName','overtake_over','SgnStartBit',0,'SgnLength',16,'SgnType','standard','ModeValue',-1,'DataType',['signed int'],'ByteLayout',['little endian'],'Factor',1,'Offset',0,'SLDataType','SS_DOUBLE'),'StatusSelected','yes','TimeSelected','no','DeltaTimeSelected','no','BytePortSelected','no','MessageLengthSelected','no','TriggerPort',struct('Selected','no','TriggerType',0),'UserCoding',struct('Selected','no','InterfaceFile','UserDecodingFile','FcnName','UserDecodeFcn','InportSelected','no','InportWidth',1,'OutportSelected','no','OutportWidth',1),'EnablePortSelected','no','UseRXService','no','BoardType','DS1','BoardNo',1,'ControllerNo',1),'OFF',[]}},'TLCFileName',{{'rtican_rx_message','OFF',[]}})  RTISFcnParameters=struct('SFcnRTICANMessage','struct','TLCFileName','char')  RTIBlockParaDefault=struct('BoardTypeNo',4302,'BoardNo',1,'ChannelNo',1,'Parameters',struct('DataFileSupport',struct('DataFileSelectedMaster',0,'DataFileSelectedLocal',0,'DataFileName','','DataFileDate','','SelectedFile',['<no file selected>']),'Options',struct('StatusSelected',1,'TimeSelected',1,'DeltaTimeSelected',1,'BytePortSelected',0,'MessageLengthSelected',0,'TriggerPort',struct('Selected',0,'TriggerType','rising'),'UserCoding',struct('Selected',0,'InterfaceFile','UserDecodingFile','FcnName','UserDecodeFcn','InportSelected',0,'InportWidth',1,'OutportSelected',0,'OutportWidth',1),'EnablePortSelected',0,'SignalOnPortnameSelected',1,'UseRXService',0),'Message',struct('MsgOnBlocknameSelected',0,'MsgName',['RX Message'],'MsgIdFormat',0,'MsgId',100,'MsgLength',8,'NumSignals',1,'SampleTime',-1,'Signal',struct('SgnName',['RX signal'],'SgnStartBit',0,'SgnLength',8,'SgnType',0,'ModeValue',-1,'DataType',0,'SLDataType','SS_DOUBLE','ByteLayout',0,'Factor',1,'Offset',0,'Min',0,'Max',255,'SgnComment',{{}},'SgnUnit',''),'MsgIdNumFormat',0,'MsgComment',{{''}}),'Version',1.2,'general',struct('isFromLib',1)),'GroupId',struct('Group',{{'RTICAN'}},'No',1,'Behavior',{{'NAMECHANGE'}},'BlockType',{{'SINK'}},'NameChangeFlag',0),'SFcnRTICANMessage',struct('MsgType','RX','MsgName',['RX Message'],'MsgIdFormat','STD','MsgId',100,'MsgLength',8,'NumSignals',1,'SampleTime',-1,'Signal',struct('SgnName',['RX signal'],'SgnStartBit',0,'SgnLength',8,'SgnType','standard','ModeValue',-1,'DataType',['unsigned int'],'ByteLayout',['little endian'],'SLDataType','SS_DOUBLE','Factor',1,'Offset',0),'StatusSelected','yes','TimeSelected','yes','DeltaTimeSelected','yes','BytePortSelected','no','MessageLengthSelected','no','EnablePortSelected','no','UserCoding',struct('Selected','no','InterfaceFile','UserDecodingFile','FcnName','UserDecodeFcn','InportSelected','no','InportWidth',1,'OutportSelected','no','OutportWidth',1),'TriggerPort',struct('Selected','no','TriggerType','rising'),'UseRXService','no','BoardType','DS4302','BoardNo',1,'ControllerNo',1,'SFcnPortType','Scalar'),'TLCFileName','rtican_rx_message')
      settings: AttributesFormatString=Group Id: RTICAN2\n  SourceProductName=dSPACE RTI CAN Blockset
  tag scope: ACC_trig=global, BBGF_Distance=global, BBGF_Speed=global, DVGF_Distance=global, GF_Distance_m=global, GF_Speed_ms=global, PCGF_Distance=global, PCGF_Speed=global, PPGF_Stop=global, PPGF_distance=global, RDGF_Distance=global, RDGF_Speed=global, Radar_distance=global, Radar_speed=global, Stop_cmd=global, System_ready=global, TouchP_start=global, TouchP_start_RX=global, color_light=global, direction_light=global, overtake_over=global
  wires:
  BBox_Geofence/1 -> Gain/1  "GF_TTC"
  BBox_Geofence/5 -> "[Disp] RX_BBox_Geofence"/1
  Gain/1 -> "[Disp] BBGF_Distance"/1, [BBGF_Distance]
  Gain5/1 -> "[Disp] BBGF_Speed"/1, [BBGF_Speed]
  BBox_Geofence/2 -> Gain5/1  "GF_Speed"
  BBox_Geofence/3 -> Gain2/1  "Nearest_X"
  BBox_Geofence/4 -> Gain3/1  "Nearest_Y"
  Gain3/1 -> "[Disp] BBGF_NearestY"/1
  Gain2/1 -> "[Disp] BBGF_NearestX"/1
  Gain8/1 -> [PCGF_Speed], "[Disp] PCGF_Speed"/1
  PCloud_Geofence/2 -> Gain8/1  "GF_Speed"
  PCloud_Geofence/1 -> Gain4/1  "GF_TTC"
  PCloud_Geofence/5 -> "[Disp] RX_PCloud_Geofence"/1
  Gain6/1 -> "[Disp] PCGF_NearestX"/1
  Gain7/1 -> "[Disp] PCGF_NearestY"/1
  PCloud_Geofence/4 -> Gain7/1  "Nearest_Y"
  Gain4/1 -> Filter/1(In1), "[Disp] PCGF_Distance_raw"/1
  PCloud_Geofence/3 -> Gain6/1  "Nearest_X"
  MATLAB Function13/3(time_out) -> "[Disp] Radar_update_gap"/1
  MATLAB Function13/2(Radar_distance_out) -> Unit Delay1/1, "[Disp] Radar_distance"/1, [Radar_distance]
  Unit Delay1/1 -> MATLAB Function13/5(Radar_distance_pre)
  Radar_Info/2 -> Gain10/1  "Radar_distance"
  Unit Delay/1 -> MATLAB Function13/4(Radar_speed_pre)
  Radar_Info/3 -> "[Disp] Radar_RX"/1, MATLAB Function13/3(Radar_RX)
  Gain10/1 -> MATLAB Function13/2(Radar_distance)
  Gain9/1 -> MATLAB Function13/1(Radar_speed)
  Radar_Info/1 -> Gain9/1  "Radar_speed"
  MATLAB Function13/1(Radar_speed_out) -> Unit Delay/1, "[Disp] Radar_speed"/1, [Radar_speed]
  Gain11/1 -> "[Disp] PPGF_Stop"/1, [PPGF_Stop]
  PP_Geofence/3 -> "[Disp] RX_PP_Geofence"/1
  Gain13/1 -> "[Disp] RDGF_NearestX"/1
  Gain14/1 -> "[Disp] RDGF_NearestY"/1
  Radar_Geofence/4 -> Gain14/1  "Nearest_Y"
  Radar_Geofence/3 -> Gain13/1  "Nearest_X"
  Radar_Geofence/2 -> Gain15/1  "GF_Speed"
  Gain15/1 -> Add/1, "[Disp] RDGF_Speed"/1
  Gain12/1 -> Switch/2, [RDGF_Distance], "[Disp] RDGF_Distance"/1
  Radar_Geofence/5 -> "[Disp] RX_BBox_Geofence1"/1
  Radar_Geofence/1 -> Gain12/1  "GF_TTC"
  [PCGF_Distance] -> Multiport Switch/3
  [BBGF_Distance] -> Multiport Switch/4
  [RDGF_Distance] -> Multiport Switch/2
  [PCGF_Speed] -> Multiport Switch1/3
  [BBGF_Speed] -> Multiport Switch1/4
  [RDGF_Speed] -> Multiport Switch1/2
  "[Para]GF_Dis_switch"/1 -> Multiport Switch/1
  Multiport Switch/1 -> "[Disp] GF_Distance"/1, Data Type Conversion1/1
  Multiport Switch1/1 -> "[Disp] GF_Speed"/1, [GF_Speed_ms]
  overtake_over/2 -> "[Disp] RX_overtake_over"/1
  "[Para]GF_Spd_switch"/1 -> Multiport Switch1/1
  [Speed_Kph] -> Gain1/1
  Gain1/1 -> Add/2
  Filter/1(Out1) -> "[Disp] PCGF_Distance"/1, [PCGF_Distance]
  MATLAB Function/1(PC_out) -> Unit Delay2/1
  Unit Delay2/1 -> MATLAB Function/3(PC_last)
  [PCGF_Distance] -> MATLAB Function/1(PC)
  [RDGF_Distance] -> MATLAB Function/2(RD)
  Compare To Constant/1 -> [ACC_trig]
  TouchP_start/1 -> [TouchP_start], "[Disp] TouchP_start"/1  "TouchP_start"
  System_ready/1 -> [System_ready], "[Disp] System_ready"/1  "System_ready"
  Stop_cmd/1 -> "[Disp] Stop_cmd1"/1, Mux/1  "Stop_01"
  Stop_cmd/2 -> "[Disp] Stop_cmd2"/1, Mux/2  "Stop_02"
  Stop_cmd/3 -> "[Disp] Stop_cmd3"/1, Mux/3  "Stop_03"
  Stop_cmd/4 -> "[Disp] Stop_cmd4"/1, Mux/4  "Stop_04"
  Stop_cmd/5 -> "[Disp] Stop_cmd5"/1, Mux/5  "Stop_05"
  Stop_cmd/6 -> "[Disp] Stop_cmd6"/1, Mux/6  "Stop_06"
  Stop_cmd/7 -> "[Disp] Stop_cmd7"/1, Mux/7  "Stop_07"
  Stop_cmd/8 -> "[Disp] Stop_cmd8"/1, Mux/8  "Stop_08"
  Mux/1 -> "[Disp] Stop_cmd"/1, [Stop_cmd]
  TouchP_start/2 -> "[Disp] TouchP_start_RX"/1, [TouchP_start_RX]
  Stop_cmd/9 -> "[Disp] Stop_cmd_RX"/1
  overtake_over/1 -> [overtake_over], "[Disp] overtake_over"/1  "overtake_over"
  Traffic_light/1 -> [color_light], "[Disp] color_light"/1  "color_light"
  Traffic_light/2 -> [direction_light], "[Disp] direction_light"/1  "direction"
  Constant/1 -> Switch/1
  Add/1 -> Switch/3
  Switch/1 -> [RDGF_Speed]
  DeviatePath_Geofence/5 -> "[Disp] RX_PCloud_Geofence1"/1
  Gain18/1 -> "[Disp] DeviatePath_NearestY"/1
  Filter1/1(Out1) -> [DVGF_Distance], "[Disp] DeviatePath_Distance"/1
  DeviatePath_Geofence/4 -> Gain18/1  "Nearest_Y"
  DeviatePath_Geofence/3 -> Gain17/1  "Nearest_X"
  Gain19/1 -> "[Disp] DeviatePath_Speed"/1
  Gain16/1 -> Filter1/1(In1), "[Disp] DeviatePath_Distance_raw"/1
  DeviatePath_Geofence/2 -> Gain19/1  "GF_Speed"
  Gain17/1 -> "[Disp] DeviatePath_NearestX"/1
  DeviatePath_Geofence/1 -> Gain16/1  "GF_distance"
  PP_Geofence/1 -> Gain11/1  "PP_stop"
  PP_Geofence/2 -> Gain20/1  "PP_distance"
  Gain20/1 -> Filter2/1(In1)
  Filter2/1(Out1) -> "[Disp] PPGF_distance"/1, [PPGF_distance]
  [DVGF_Distance] -> Switch4/1
  Constant5/1 -> Switch4/3
  "[Para]DV_enable"/1 -> Switch4/2
  Switch4/1 -> Data Type Conversion/1
  Data Type Conversion/1 -> Min/1
  Data Type Conversion1/1 -> Min/2
  Min/1 -> Compare To Constant/1, [GF_Distance_m]
